simulink library "outp"  (R2021b)
(part 11 of 11)

  VSYS_PmicBootPath_raw32_Inproc/1 -> UnitConverter707/1
  UnitConverter707/1 -> VOUTP_PmicBootPath_raw32/1  "VOUTP_PmicBootPath_raw32"
  VSYS_DrivingMode_cnt/1 -> VSYS_DrivingMode_cnt_Inproc/1  "VSYS_DrivingMode_cnt"
  VSYS_DrivingMode_cnt_Inproc/1 -> UnitConverter708/1
  UnitConverter708/1 -> VOUTP_DrivingMode_cnt/1  "VOUTP_DrivingMode_cnt"
  VSYS_ModelYear_cnt/1 -> VSYS_ModelYear_cnt_Inproc/1  "VSYS_ModelYear_cnt"
  VSYS_ModelYear_cnt_Inproc/1 -> UnitConverter709/1
  UnitConverter709/1 -> VOUTP_ModelYear_cnt/1  "VOUTP_ModelYear_cnt"
  VSYS_Var4_cnt/1 -> VSYS_Var4_cnt_Inproc/1  "VSYS_Var4_cnt"
  VSYS_Var4_cnt_Inproc/1 -> UnitConverter710/1
  UnitConverter710/1 -> VOUTP_Var4_cnt/1  "VOUTP_Var4_cnt"
  VSYS_Var5_cnt/1 -> VSYS_Var5_cnt_Inproc/1  "VSYS_Var5_cnt"
  VSYS_Var5_cnt_Inproc/1 -> UnitConverter711/1
  UnitConverter711/1 -> VOUTP_Var5_cnt/1  "VOUTP_Var5_cnt"
  VTHC_FDCompCmd_rpm/1 -> VTHC_FDCompCmd_rpm_Inproc/1  "VTHC_FDCompCmd_rpm"
  VTHC_FDCompCmd_rpm_Inproc/1 -> UnitConverter712/1
  UnitConverter712/1 -> VOUTP_FDCompCmd_rpm/1  "VOUTP_FDCompCmd_rpm"
  VTHC_FDSOV1Cmd_flg/1 -> VTHC_FDSOV1Cmd_flg_Inproc/1  "VTHC_FDSOV1Cmd_flg"
  VTHC_FDSOV1Cmd_flg_Inproc/1 -> UnitConverter713/1
  UnitConverter713/1 -> VOUTP_FDSOV1Cmd_flg/1  "VOUTP_FDSOV1Cmd_flg"
  VTHC_FDSOV2Cmd_flg/1 -> VTHC_FDSOV2Cmd_flg_Inproc/1  "VTHC_FDSOV2Cmd_flg"
  VTHC_FDSOV2Cmd_flg_Inproc/1 -> UnitConverter714/1
  UnitConverter714/1 -> VOUTP_FDSOV2Cmd_flg/1  "VOUTP_FDSOV2Cmd_flg"
  VTHC_FDSOV3Cmd_flg/1 -> VTHC_FDSOV3Cmd_flg_Inproc/1  "VTHC_FDSOV3Cmd_flg"
  VTHC_FDSOV3Cmd_flg_Inproc/1 -> UnitConverter715/1
  UnitConverter715/1 -> VOUTP_FDSOV3Cmd_flg/1  "VOUTP_FDSOV3Cmd_flg"
  VTHC_FDEXV1Cmd_step/1 -> VTHC_FDEXV1Cmd_step_Inproc/1  "VTHC_FDEXV1Cmd_step"
  VTHC_FDEXV1Cmd_step_Inproc/1 -> UnitConverter716/1
  UnitConverter716/1 -> VOUTP_FDEXV1Cmd_step/1  "VOUTP_FDEXV1Cmd_step"
  VTHC_FDEXV2Cmd_step/1 -> VTHC_FDEXV2Cmd_step_Inproc/1  "VTHC_FDEXV2Cmd_step"
  VTHC_FDEXV2Cmd_step_Inproc/1 -> UnitConverter717/1
  UnitConverter717/1 -> VOUTP_FDEXV2Cmd_step/1  "VOUTP_FDEXV2Cmd_step"
  VTHC_FDSOTXVCmd_flg/1 -> VTHC_FDSOTXVCmd_flg_Inproc/1  "VTHC_FDSOTXVCmd_flg"
  VTHC_FDSOTXVCmd_flg_Inproc/1 -> UnitConverter718/1
  UnitConverter718/1 -> VOUTP_FDSOTXVCmd_flg/1  "VOUTP_FDSOTXVCmd_flg"
  VTHC_FDFWVCmd_flg/1 -> VTHC_FDFWVCmd_flg_Inproc/1  "VTHC_FDFWVCmd_flg"
  VTHC_FDFWVCmd_flg_Inproc/1 -> UnitConverter719/1
  UnitConverter719/1 -> VOUTP_FDFWVCmd_flg/1  "VOUTP_FDFWVCmd_flg"
  VTHC_FDTWVCmd_pct/1 -> VTHC_FDTWVCmd_pct_Inproc/1  "VTHC_FDTWVCmd_pct"
  VTHC_FDTWVCmd_pct_Inproc/1 -> UnitConverter720/1
  UnitConverter720/1 -> VOUTP_FDTWVCmd_pct/1  "VOUTP_FDTWVCmd_pct"
  VTHC_FDFrWPTCHeatPwrCmd_W/1 -> VTHC_FDFrWPTCHeatPwrCmd_W_Inproc/1  "VTHC_FDFrWPTCHeatPwrCmd_W"
  VTHC_FDFrWPTCHeatPwrCmd_W_Inproc/1 -> UnitConverter721/1
  UnitConverter721/1 -> VOUTP_FDFrWPTCHeatPwrCmd_W/1  "VOUTP_FDFrWPTCHeatPwrCmd_W"
  VTHC_CoolgFanActDuty_pct/1 -> VTHC_CoolgFanActDuty_pct_Inproc/1  "VTHC_CoolgFanActDuty_pct"
  VTHC_CoolgFanActDuty_pct_Inproc/1 -> UnitConverter722/1
  UnitConverter722/1 -> VOUTP_CoolgFanActDuty_pct/1  "VOUTP_CoolgFanActDuty_pct"
  VTHC_FDAGSCmd_enum/1 -> VTHC_FDAGSCmd_enum_Inproc/1  "VTHC_FDAGSCmd_enum"
  VTHC_FDAGSCmd_enum_Inproc/1 -> UnitConverter723/1
  UnitConverter723/1 -> VOUTP_FDAGSCmd_enum/1  "VOUTP_FDAGSCmd_enum"
  VTHC_FDEWP1Cmd_enum/1 -> VTHC_FDEWP1Cmd_enum_Inproc/1  "VTHC_FDEWP1Cmd_enum"
  VTHC_FDEWP1Cmd_enum_Inproc/1 -> UnitConverter724/1
  UnitConverter724/1 -> VOUTP_FDEWP1Cmd_enum/1  "VOUTP_FDEWP1Cmd_enum"
  VTHC_FDEWP2Cmd_enum/1 -> VTHC_FDEWP2Cmd_enum_Inproc/1  "VTHC_FDEWP2Cmd_enum"
  VTHC_FDEWP2Cmd_enum_Inproc/1 -> UnitConverter725/1
  UnitConverter725/1 -> VOUTP_FDEWP2Cmd_enum/1  "VOUTP_FDEWP2Cmd_enum"
  VTHC_FDEWP3Cmd_enum/1 -> VTHC_FDEWP3Cmd_enum_Inproc/1  "VTHC_FDEWP3Cmd_enum"
  VTHC_FDEWP3Cmd_enum_Inproc/1 -> UnitConverter726/1
  UnitConverter726/1 -> VOUTP_FDEWP3Cmd_enum/1  "VOUTP_FDEWP3Cmd_enum"
  VTHC_FDFrLeAPTCHeatPwrCmd_W/1 -> VTHC_FDFrLeAPTCHeatPwrCmd_W_Inproc/1  "VTHC_FDFrLeAPTCHeatPwrCmd_W"
  VTHC_FDFrLeAPTCHeatPwrCmd_W_Inproc/1 -> UnitConverter727/1
  UnitConverter727/1 -> VOUTP_FDFrLeAPTCHeatPwrCmd_W/1  "VOUTP_FDFrLeAPTCHeatPwrCmd_W"
  VTHC_FDFrRiAPTCHeatPwrCmd_W/1 -> VTHC_FDFrRiAPTCHeatPwrCmd_W_Inproc/1  "VTHC_FDFrRiAPTCHeatPwrCmd_W"
  VTHC_FDFrRiAPTCHeatPwrCmd_W_Inproc/1 -> UnitConverter728/1
  UnitConverter728/1 -> VOUTP_FDFrRiAPTCHeatPwrCmd_W/1  "VOUTP_FDFrRiAPTCHeatPwrCmd_W"
  VTHC_FDRrAPTCHeatPwrCmd_W/1 -> VTHC_FDRrAPTCHeatPwrCmd_W_Inproc/1  "VTHC_FDRrAPTCHeatPwrCmd_W"
  VTHC_FDRrAPTCHeatPwrCmd_W_Inproc/1 -> UnitConverter729/1
  UnitConverter729/1 -> VOUTP_FDRrAPTCHeatPwrCmd_W/1  "VOUTP_FDRrAPTCHeatPwrCmd_W"
  VTHC_FDBlowerCmd_pct/1 -> VTHC_FDBlowerCmd_pct_Inproc/1  "VTHC_FDBlowerCmd_pct"
  VTHC_FDBlowerCmd_pct_Inproc/1 -> UnitConverter730/1
  UnitConverter730/1 -> VOUTP_FDBlowerCmd_pct/1  "VOUTP_FDBlowerCmd_pct"
  VTHC_BatteryMode_enum/1 -> VTHC_BatteryMode_enum_Inproc/1  "VTHC_BatteryMode_enum"
  VTHC_BatteryMode_enum_Inproc/1 -> UnitConverter731/1
  UnitConverter731/1 -> VOUTP_BatteryMode_enum/1  "VOUTP_BatteryMode_enum"
  VTHC_EDriveMode_enum/1 -> VTHC_EDriveMode_enum_Inproc/1  "VTHC_EDriveMode_enum"
  VTHC_EDriveMode_enum_Inproc/1 -> UnitConverter732/1
  UnitConverter732/1 -> VOUTP_EDriveMode_enum/1  "VOUTP_EDriveMode_enum"
  VTHC_CabinMode_enum/1 -> VTHC_CabinMode_enum_Inproc/1  "VTHC_CabinMode_enum"
  VTHC_CabinMode_enum_Inproc/1 -> UnitConverter733/1
  UnitConverter733/1 -> VOUTP_CabinMode_enum/1  "VOUTP_CabinMode_enum"
  VTHC_CCUACLampSts_flg/1 -> VTHC_CCUACLampSts_flg_Inproc/1  "VTHC_CCUACLampSts_flg"
  VTHC_CCUACLampSts_flg_Inproc/1 -> UnitConverter734/1
  UnitConverter734/1 -> VOUTP_CCUACLampSts_flg/1  "VOUTP_CCUACLampSts_flg"
  VTHC_CCUAutoLampSts_flg/1 -> VTHC_CCUAutoLampSts_flg_Inproc/1  "VTHC_CCUAutoLampSts_flg"
  VTHC_CCUAutoLampSts_flg_Inproc/1 -> UnitConverter735/1
  UnitConverter735/1 -> VOUTP_CCUAutoLampSts_flg/1  "VOUTP_CCUAutoLampSts_flg"
  VTHC_CCUACMaxLampSts_flg/1 -> VTHC_CCUACMaxLampSts_flg_Inproc/1  "VTHC_CCUACMaxLampSts_flg"
  VTHC_CCUACMaxLampSts_flg_Inproc/1 -> UnitConverter736/1
  UnitConverter736/1 -> VOUTP_CCUACMaxLampSts_flg/1  "VOUTP_CCUACMaxLampSts_flg"
  VTHC_CCUSyncLampSts_flg/1 -> VTHC_CCUSyncLampSts_flg_Inproc/1  "VTHC_CCUSyncLampSts_flg"
  VTHC_CCUSyncLampSts_flg_Inproc/1 -> UnitConverter737/1
  UnitConverter737/1 -> VOUTP_CCUSyncLampSts_flg/1  "VOUTP_CCUSyncLampSts_flg"
  VTHC_sigAirIntenZon1St_enum/1 -> VTHC_sigAirIntenZon1St_enum_Inproc/1  "VTHC_sigAirIntenZon1St_enum"
  VTHC_sigAirIntenZon1St_enum_Inproc/1 -> UnitConverter738/1
  UnitConverter738/1 -> VOUTP_sigAirIntenZon1St_enum/1  "VOUTP_sigAirIntenZon1St_enum"
  VTHC_sigWindDirZon1St_enum/1 -> VTHC_sigWindDirZon1St_enum_Inproc/1  "VTHC_sigWindDirZon1St_enum"
  VTHC_sigWindDirZon1St_enum_Inproc/1 -> UnitConverter739/1
  UnitConverter739/1 -> VOUTP_sigWindDirZon1St_enum/1  "VOUTP_sigWindDirZon1St_enum"
  VTHC_sigRecircSt_flg/1 -> VTHC_sigRecircSt_flg_Inproc/1  "VTHC_sigRecircSt_flg"
  VTHC_sigRecircSt_flg_Inproc/1 -> UnitConverter740/1
  UnitConverter740/1 -> VOUTP_sigRecircSt_flg/1  "VOUTP_sigRecircSt_flg"
  VTHC_sigSetTempZon1St_C/1 -> VTHC_sigSetTempZon1St_C_Inproc/1  "VTHC_sigSetTempZon1St_C"
  VTHC_sigSetTempZon1St_C_Inproc/1 -> UnitConverter741/1
  UnitConverter741/1 -> VOUTP_sigSetTempZon1St_C/1  "VOUTP_sigSetTempZon1St_C"
  VTHC_sigSetTempZon2St_C/1 -> VTHC_sigSetTempZon2St_C_Inproc/1  "VTHC_sigSetTempZon2St_C"
  VTHC_sigSetTempZon2St_C_Inproc/1 -> UnitConverter742/1
  UnitConverter742/1 -> VOUTP_sigSetTempZon2St_C/1  "VOUTP_sigSetTempZon2St_C"
  VTHC_sigClntTHvBattOut_C/1 -> VTHC_sigClntTHvBattOut_C_Inproc/1  "VTHC_sigClntTHvBattOut_C"
  VTHC_sigClntTHvBattOut_C_Inproc/1 -> UnitConverter743/1
  UnitConverter743/1 -> VOUTP_sigClntTHvBattOut_C/1  "VOUTP_sigClntTHvBattOut_C"
  VTHC_sigCbnSolarLeft_W/1 -> VTHC_sigCbnSolarLeft_W_Inproc/1  "VTHC_sigCbnSolarLeft_W"
  VTHC_sigCbnSolarLeft_W_Inproc/1 -> UnitConverter744/1
  UnitConverter744/1 -> VOUTP_sigCbnSolarLeft_W/1  "VOUTP_sigCbnSolarLeft_W"
  VTHC_sigClntTHvBattIn_C/1 -> VTHC_sigClntTHvBattIn_C_Inproc/1  "VTHC_sigClntTHvBattIn_C"
  VTHC_sigClntTHvBattIn_C_Inproc/1 -> UnitConverter745/1
  UnitConverter745/1 -> VOUTP_sigClntTHvBattIn_C/1  "VOUTP_sigClntTHvBattIn_C"
  VTHC_sigCbnSolarRight_W/1 -> VTHC_sigCbnSolarRight_W_Inproc/1  "VTHC_sigCbnSolarRight_W"
  VTHC_sigCbnSolarRight_W_Inproc/1 -> UnitConverter746/1
  UnitConverter746/1 -> VOUTP_sigCbnSolarRight_W/1  "VOUTP_sigCbnSolarRight_W"
  VTHC_sigAmbAirT_C/1 -> VTHC_sigAmbAirT_C_Inproc/1  "VTHC_sigAmbAirT_C"
  VTHC_sigAmbAirT_C_Inproc/1 -> UnitConverter747/1
  UnitConverter747/1 -> VOUTP_sigAmbAirT_C/1  "VOUTP_sigAmbAirT_C"
  VTHC_sigCbnAirT_C/1 -> VTHC_sigCbnAirT_C_Inproc/1  "VTHC_sigCbnAirT_C"
  VTHC_sigCbnAirT_C_Inproc/1 -> UnitConverter748/1
  UnitConverter748/1 -> VOUTP_sigCbnAirT_C/1  "VOUTP_sigCbnAirT_C"
  VTHC_ACSubMode_enum/1 -> VTHC_ACSubMode_enum_Inproc/1  "VTHC_ACSubMode_enum"
  VTHC_ACSubMode_enum_Inproc/1 -> UnitConverter749/1
  UnitConverter749/1 -> VOUTP_ACSubMode_enum/1  "VOUTP_ACSubMode_enum"
  VTHC_FDRecyAutoCmd_enum/1 -> VTHC_FDRecyAutoCmd_enum_Inproc/1  "VTHC_FDRecyAutoCmd_enum"
  VTHC_FDRecyAutoCmd_enum_Inproc/1 -> UnitConverter750/1
  UnitConverter750/1 -> VOUTP_FDRecyAutoCmd_enum/1  "VOUTP_FDRecyAutoCmd_enum"
  VTHC_ACModeMem_enum/1 -> VTHC_ACModeMem_enum_Inproc/1  "VTHC_ACModeMem_enum"
  VTHC_ACModeMem_enum_Inproc/1 -> UnitConverter751/1
  UnitConverter751/1 -> VOUTP_ACModeMem_enum/1  "VOUTP_ACModeMem_enum"
  VTHC_Face_flg/1 -> VTHC_Face_flg_Inproc/1  "VTHC_Face_flg"
  VTHC_Face_flg_Inproc/1 -> UnitConverter752/1
  UnitConverter752/1 -> VOUTP_Face_flg/1  "VOUTP_Face_flg"
  VTHC_Foot_flg/1 -> VTHC_Foot_flg_Inproc/1  "VTHC_Foot_flg"
  VTHC_Foot_flg_Inproc/1 -> UnitConverter753/1
  UnitConverter753/1 -> VOUTP_Foot_flg/1  "VOUTP_Foot_flg"
  VTHC_Frost_flg/1 -> VTHC_Frost_flg_Inproc/1  "VTHC_Frost_flg"
  VTHC_Frost_flg_Inproc/1 -> UnitConverter754/1
  UnitConverter754/1 -> VOUTP_Frost_flg/1  "VOUTP_Frost_flg"
  VTHC_FaceM_flg/1 -> VTHC_FaceM_flg_Inproc/1  "VTHC_FaceM_flg"
  VTHC_FaceM_flg_Inproc/1 -> UnitConverter755/1
  UnitConverter755/1 -> VOUTP_FaceM_flg/1  "VOUTP_FaceM_flg"
  VTHC_FootM_flg/1 -> VTHC_FootM_flg_Inproc/1  "VTHC_FootM_flg"
  VTHC_FootM_flg_Inproc/1 -> UnitConverter756/1
  UnitConverter756/1 -> VOUTP_FootM_flg/1  "VOUTP_FootM_flg"
  VTHC_CCUSyncSts_flg/1 -> VTHC_CCUSyncSts_flg_Inproc/1  "VTHC_CCUSyncSts_flg"
  VTHC_CCUSyncSts_flg_Inproc/1 -> UnitConverter757/1
  UnitConverter757/1 -> VOUTP_CCUSyncSts_flg/1  "VOUTP_CCUSyncSts_flg"
  VTHC_ACForceOFF_flg/1 -> VTHC_ACForceOFF_flg_Inproc/1  "VTHC_ACForceOFF_flg"
  VTHC_ACForceOFF_flg_Inproc/1 -> UnitConverter758/1
  UnitConverter758/1 -> VOUTP_ACForceOFF_flg/1  "VOUTP_ACForceOFF_flg"
  VTHC_RecAutoFlg_flg/1 -> VTHC_RecAutoFlg_flg_Inproc/1  "VTHC_RecAutoFlg_flg"
  VTHC_RecAutoFlg_flg_Inproc/1 -> UnitConverter759/1
  UnitConverter759/1 -> VOUTP_RecAutoFlg_flg/1  "VOUTP_RecAutoFlg_flg"
  VTHC_AirIntenZone1M_enum/1 -> VTHC_AirIntenZone1M_enum_Inproc/1  "VTHC_AirIntenZone1M_enum"
  VTHC_AirIntenZone1M_enum_Inproc/1 -> UnitConverter760/1
  UnitConverter760/1 -> VOUTP_AirIntenZone1M_enum/1  "VOUTP_AirIntenZone1M_enum"
  VTHC_fdefog_flg/1 -> VTHC_fdefog_flg_Inproc/1  "VTHC_fdefog_flg"
  VTHC_fdefog_flg_Inproc/1 -> UnitConverter761/1
  UnitConverter761/1 -> VOUTP_fdefog_flg/1  "VOUTP_fdefog_flg"
  VTHC_sigSetTempZon2StM_C/1 -> VTHC_sigSetTempZon2StM_C_Inproc/1  "VTHC_sigSetTempZon2StM_C"
  VTHC_sigSetTempZon2StM_C_Inproc/1 -> UnitConverter762/1
  UnitConverter762/1 -> VOUTP_sigSetTempZon2StM_C/1  "VOUTP_sigSetTempZon2StM_C"
  VTHC_sigDfrstSt_flg/1 -> VTHC_sigDfrstSt_flg_Inproc/1  "VTHC_sigDfrstSt_flg"
  VTHC_sigDfrstSt_flg_Inproc/1 -> UnitConverter763/1
  UnitConverter763/1 -> VOUTP_sigDfrstSt_flg/1  "VOUTP_sigDfrstSt_flg"
  VTHC_FDCTHCAirIntZ3Sta_enum/1 -> VTHC_FDCTHCAirIntZ3Sta_enum_Inproc/1  "VTHC_FDCTHCAirIntZ3Sta_enum"
  VTHC_FDCTHCAirIntZ3Sta_enum_Inproc/1 -> UnitConverter764/1
  UnitConverter764/1 -> VOUTP_FDCTHCAirIntZ3Sta_enum/1  "VOUTP_FDCTHCAirIntZ3Sta_enum"
  VTHC_FDCTHCLEVentModeSta_enum/1 -> VTHC_FDCTHCLEVentModeSta_enum_Inproc/1  "VTHC_FDCTHCLEVentModeSta_enum"
  VTHC_FDCTHCLEVentModeSta_enum_Inproc/1 -> UnitConverter765/1
  UnitConverter765/1 -> VOUTP_FDCTHCLEVentModeSta_enum/1  "VOUTP_FDCTHCLEVentModeSta_enum"
  VTHC_FDCTHCREVentModeSta_enum/1 -> VTHC_FDCTHCREVentModeSta_enum_Inproc/1  "VTHC_FDCTHCREVentModeSta_enum"
  VTHC_FDCTHCREVentModeSta_enum_Inproc/1 -> UnitConverter766/1
  UnitConverter766/1 -> VOUTP_FDCTHCREVentModeSta_enum/1  "VOUTP_FDCTHCREVentModeSta_enum"
  VTHC_FDCTHCLEVentZSta_enum/1 -> VTHC_FDCTHCLEVentZSta_enum_Inproc/1  "VTHC_FDCTHCLEVentZSta_enum"
  VTHC_FDCTHCLEVentZSta_enum_Inproc/1 -> UnitConverter767/1
  UnitConverter767/1 -> VOUTP_FDCTHCLEVentZSta_enum/1  "VOUTP_FDCTHCLEVentZSta_enum"
  VTHC_FDCTHCCLEVentZSta_enum/1 -> VTHC_FDCTHCCLEVentZSta_enum_Inproc/1  "VTHC_FDCTHCCLEVentZSta_enum"
  VTHC_FDCTHCCLEVentZSta_enum_Inproc/1 -> UnitConverter768/1
  UnitConverter768/1 -> VOUTP_FDCTHCCLEVentZSta_enum/1  "VOUTP_FDCTHCCLEVentZSta_enum"
  VTHC_FDCTHCREVentZSta_enum/1 -> VTHC_FDCTHCREVentZSta_enum_Inproc/1  "VTHC_FDCTHCREVentZSta_enum"
  VTHC_FDCTHCREVentZSta_enum_Inproc/1 -> UnitConverter769/1
  UnitConverter769/1 -> VOUTP_FDCTHCREVentZSta_enum/1  "VOUTP_FDCTHCREVentZSta_enum"
  VTHC_FDCTHCCREVentZSta_enum/1 -> VTHC_FDCTHCCREVentZSta_enum_Inproc/1  "VTHC_FDCTHCCREVentZSta_enum"
  VTHC_FDCTHCCREVentZSta_enum_Inproc/1 -> UnitConverter770/1
  UnitConverter770/1 -> VOUTP_FDCTHCCREVentZSta_enum/1  "VOUTP_FDCTHCCREVentZSta_enum"
  VTHC_FDCTHCLEVentYSta_enum/1 -> VTHC_FDCTHCLEVentYSta_enum_Inproc/1  "VTHC_FDCTHCLEVentYSta_enum"
  VTHC_FDCTHCLEVentYSta_enum_Inproc/1 -> UnitConverter771/1
  UnitConverter771/1 -> VOUTP_FDCTHCLEVentYSta_enum/1  "VOUTP_FDCTHCLEVentYSta_enum"
  VTHC_FDCTHCLVentENSta_flg/1 -> VTHC_FDCTHCLVentENSta_flg_Inproc/1  "VTHC_FDCTHCLVentENSta_flg"
  VTHC_FDCTHCLVentENSta_flg_Inproc/1 -> UnitConverter772/1
  UnitConverter772/1 -> VOUTP_FDCTHCLVentENSta_flg/1  "VOUTP_FDCTHCLVentENSta_flg"
  VTHC_FDCTHCCLEVentYSta_enum/1 -> VTHC_FDCTHCCLEVentYSta_enum_Inproc/1  "VTHC_FDCTHCCLEVentYSta_enum"
  VTHC_FDCTHCCLEVentYSta_enum_Inproc/1 -> UnitConverter773/1
  UnitConverter773/1 -> VOUTP_FDCTHCCLEVentYSta_enum/1  "VOUTP_FDCTHCCLEVentYSta_enum"
  VTHC_FDCTHCCLVentENSta_flg/1 -> VTHC_FDCTHCCLVentENSta_flg_Inproc/1  "VTHC_FDCTHCCLVentENSta_flg"
  VTHC_FDCTHCCLVentENSta_flg_Inproc/1 -> UnitConverter774/1
  UnitConverter774/1 -> VOUTP_FDCTHCCLVentENSta_flg/1  "VOUTP_FDCTHCCLVentENSta_flg"
  VTHC_FDCTHCREVentYSta_enum/1 -> VTHC_FDCTHCREVentYSta_enum_Inproc/1  "VTHC_FDCTHCREVentYSta_enum"
  VTHC_FDCTHCREVentYSta_enum_Inproc/1 -> UnitConverter775/1
  UnitConverter775/1 -> VOUTP_FDCTHCREVentYSta_enum/1  "VOUTP_FDCTHCREVentYSta_enum"
  VTHC_FDCTHCRVentENSta_flg/1 -> VTHC_FDCTHCRVentENSta_flg_Inproc/1  "VTHC_FDCTHCRVentENSta_flg"
  VTHC_FDCTHCRVentENSta_flg_Inproc/1 -> UnitConverter776/1
  UnitConverter776/1 -> VOUTP_FDCTHCRVentENSta_flg/1  "VOUTP_FDCTHCRVentENSta_flg"
  VTHC_FDCTHCCREVentYSta_enum/1 -> VTHC_FDCTHCCREVentYSta_enum_Inproc/1  "VTHC_FDCTHCCREVentYSta_enum"
  VTHC_FDCTHCCREVentYSta_enum_Inproc/1 -> UnitConverter777/1
  UnitConverter777/1 -> VOUTP_FDCTHCCREVentYSta_enum/1  "VOUTP_FDCTHCCREVentYSta_enum"
  VTHC_FDCTHCCRVentENSta_flg/1 -> VTHC_FDCTHCCRVentENSta_flg_Inproc/1  "VTHC_FDCTHCCRVentENSta_flg"
  VTHC_FDCTHCCRVentENSta_flg_Inproc/1 -> UnitConverter778/1
  UnitConverter778/1 -> VOUTP_FDCTHCCRVentENSta_flg/1  "VOUTP_FDCTHCCRVentENSta_flg"
  VTHC_FDCTHCMAPTCForceOFFSta_flg/1 -> VTHC_FDCTHCMAPTCForceOFFSta_flg_Inproc/1  "VTHC_FDCTHCMAPTCForceOFFSta_flg"
  VTHC_FDCTHCMAPTCForceOFFSta_flg_Inproc/1 -> UnitConverter779/1
  UnitConverter779/1 -> VOUTP_FDCTHCMAPTCForceOFFSta_flg/1  "VOUTP_FDCTHCMAPTCForceOFFSta_flg"
  VTHC_FDCFGSAirIntSta_enum/1 -> VTHC_FDCFGSAirIntSta_enum_Inproc/1  "VTHC_FDCFGSAirIntSta_enum"
  VTHC_FDCFGSAirIntSta_enum_Inproc/1 -> UnitConverter780/1
  UnitConverter780/1 -> VOUTP_FDCFGSAirIntSta_enum/1  "VOUTP_FDCFGSAirIntSta_enum"
  VTHC_FDCFGSChSta_enum/1 -> VTHC_FDCFGSChSta_enum_Inproc/1  "VTHC_FDCFGSChSta_enum"
  VTHC_FDCFGSChSta_enum_Inproc/1 -> UnitConverter781/1
  UnitConverter781/1 -> VOUTP_FDCFGSChSta_enum/1  "VOUTP_FDCFGSChSta_enum"
  VTHC_FDCFGSAirIntCmd_enum/1 -> VTHC_FDCFGSAirIntCmd_enum_Inproc/1  "VTHC_FDCFGSAirIntCmd_enum"
  VTHC_FDCFGSAirIntCmd_enum_Inproc/1 -> UnitConverter782/1
  UnitConverter782/1 -> VOUTP_FDCFGSAirIntCmd_enum/1  "VOUTP_FDCFGSAirIntCmd_enum"
  VTHC_FDCFGSFuncSta_enum/1 -> VTHC_FDCFGSFuncSta_enum_Inproc/1  "VTHC_FDCFGSFuncSta_enum"
  VTHC_FDCFGSFuncSta_enum_Inproc/1 -> UnitConverter783/1
  UnitConverter783/1 -> VOUTP_FDCFGSFuncSta_enum/1  "VOUTP_FDCFGSFuncSta_enum"
  VTHC_FDCFGSChCmd_enum/1 -> VTHC_FDCFGSChCmd_enum_Inproc/1  "VTHC_FDCFGSChCmd_enum"
  VTHC_FDCFGSChCmd_enum_Inproc/1 -> UnitConverter784/1
  UnitConverter784/1 -> VOUTP_FDCFGSChCmd_enum/1  "VOUTP_FDCFGSChCmd_enum"
  VTHC_FDCFGSIONSWSta_flg/1 -> VTHC_FDCFGSIONSWSta_flg_Inproc/1  "VTHC_FDCFGSIONSWSta_flg"
  VTHC_FDCFGSIONSWSta_flg_Inproc/1 -> UnitConverter785/1
  UnitConverter785/1 -> VOUTP_FDCFGSIONSWSta_flg/1  "VOUTP_FDCFGSIONSWSta_flg"
  VTHC_FDCFGSIONCmd_flg/1 -> VTHC_FDCFGSIONCmd_flg_Inproc/1  "VTHC_FDCFGSIONCmd_flg"
  VTHC_FDCFGSIONCmd_flg_Inproc/1 -> UnitConverter786/1
  UnitConverter786/1 -> VOUTP_FDCFGSIONCmd_flg/1  "VOUTP_FDCFGSIONCmd_flg"
  VTHC_FDCTHCMPreWPTCHeatSta_enum/1 -> VTHC_FDCTHCMPreWPTCHeatSta_enum_Inproc/1  "VTHC_FDCTHCMPreWPTCHeatSta_enum"
  VTHC_FDCTHCMPreWPTCHeatSta_enum_Inproc/1 -> UnitConverter787/1
  UnitConverter787/1 -> VOUTP_FDCTHCMPreWPTCHeatSta_enum/1  "VOUTP_FDCTHCMPreWPTCHeatSta_enum"
  VTHC_EWPBUflag1_flg/1 -> VTHC_EWPBUflag1_flg_Inproc/1  "VTHC_EWPBUflag1_flg"
  VTHC_EWPBUflag1_flg_Inproc/1 -> UnitConverter788/1
  UnitConverter788/1 -> VOUTP_EWPBUflag1_flg/1  "VOUTP_EWPBUflag1_flg"
  VTHC_EWPBUflag2_flg/1 -> VTHC_EWPBUflag2_flg_Inproc/1  "VTHC_EWPBUflag2_flg"
  VTHC_EWPBUflag2_flg_Inproc/1 -> UnitConverter789/1
  UnitConverter789/1 -> VOUTP_EWPBUflag2_flg/1  "VOUTP_EWPBUflag2_flg"
  VTHC_EWPBUflag3_flg/1 -> VTHC_EWPBUflag3_flg_Inproc/1  "VTHC_EWPBUflag3_flg"
  VTHC_EWPBUflag3_flg_Inproc/1 -> UnitConverter790/1
  UnitConverter790/1 -> VOUTP_EWPBUflag3_flg/1  "VOUTP_EWPBUflag3_flg"
  VTHC_FaceMSet_enum/1 -> VTHC_FaceMSet_enum_Inproc/1  "VTHC_FaceMSet_enum"
  VTHC_FaceMSet_enum_Inproc/1 -> UnitConverter791/1
  UnitConverter791/1 -> VOUTP_FaceMSet_enum/1  "VOUTP_FaceMSet_enum"
  VTHC_FootMSet_enum/1 -> VTHC_FootMSet_enum_Inproc/1  "VTHC_FootMSet_enum"
  VTHC_FootMSet_enum_Inproc/1 -> UnitConverter792/1
  UnitConverter792/1 -> VOUTP_FootMSet_enum/1  "VOUTP_FootMSet_enum"
  VTHC_fdefogSet_enum/1 -> VTHC_fdefogSet_enum_Inproc/1  "VTHC_fdefogSet_enum"
  VTHC_fdefogSet_enum_Inproc/1 -> UnitConverter793/1
  UnitConverter793/1 -> VOUTP_fdefogSet_enum/1  "VOUTP_fdefogSet_enum"
  VTHC_CCUSyncStsSet_enum/1 -> VTHC_CCUSyncStsSet_enum_Inproc/1  "VTHC_CCUSyncStsSet_enum"
  VTHC_CCUSyncStsSet_enum_Inproc/1 -> UnitConverter794/1
  UnitConverter794/1 -> VOUTP_CCUSyncStsSet_enum/1  "VOUTP_CCUSyncStsSet_enum"
  VTHC_sigRecircStSet_enum/1 -> VTHC_sigRecircStSet_enum_Inproc/1  "VTHC_sigRecircStSet_enum"
  VTHC_sigRecircStSet_enum_Inproc/1 -> UnitConverter795/1
  UnitConverter795/1 -> VOUTP_sigRecircStSet_enum/1  "VOUTP_sigRecircStSet_enum"
  VTHC_RecyAutoSet_enum/1 -> VTHC_RecyAutoSet_enum_Inproc/1  "VTHC_RecyAutoSet_enum"
  VTHC_RecyAutoSet_enum_Inproc/1 -> UnitConverter796/1
  UnitConverter796/1 -> VOUTP_RecyAutoSet_enum/1  "VOUTP_RecyAutoSet_enum"
  VTHC_AirIntenZone1MSet1_enum/1 -> VTHC_AirIntenZone1MSet1_enum_Inproc/1  "VTHC_AirIntenZone1MSet1_enum"
  VTHC_AirIntenZone1MSet1_enum_Inproc/1 -> UnitConverter797/1
  UnitConverter797/1 -> VOUTP_AirIntenZone1MSet1_enum/1  "VOUTP_AirIntenZone1MSet1_enum"
  VTHC_AirIntenZone1MSet2_enum/1 -> VTHC_AirIntenZone1MSet2_enum_Inproc/1  "VTHC_AirIntenZone1MSet2_enum"
  VTHC_AirIntenZone1MSet2_enum_Inproc/1 -> UnitConverter798/1
  UnitConverter798/1 -> VOUTP_AirIntenZone1MSet2_enum/1  "VOUTP_AirIntenZone1MSet2_enum"
  VTHC_AirIntenZone1MSet3_enum/1 -> VTHC_AirIntenZone1MSet3_enum_Inproc/1  "VTHC_AirIntenZone1MSet3_enum"
  VTHC_AirIntenZone1MSet3_enum_Inproc/1 -> UnitConverter799/1
  UnitConverter799/1 -> VOUTP_AirIntenZone1MSet3_enum/1  "VOUTP_AirIntenZone1MSet3_enum"
  VTHC_AirIntenZone1MSet4_enum/1 -> VTHC_AirIntenZone1MSet4_enum_Inproc/1  "VTHC_AirIntenZone1MSet4_enum"
  VTHC_AirIntenZone1MSet4_enum_Inproc/1 -> UnitConverter800/1
  UnitConverter800/1 -> VOUTP_AirIntenZone1MSet4_enum/1  "VOUTP_AirIntenZone1MSet4_enum"
  VTHC_AirIntenZone1MSet5_enum/1 -> VTHC_AirIntenZone1MSet5_enum_Inproc/1  "VTHC_AirIntenZone1MSet5_enum"
  VTHC_AirIntenZone1MSet5_enum_Inproc/1 -> UnitConverter801/1
  UnitConverter801/1 -> VOUTP_AirIntenZone1MSet5_enum/1  "VOUTP_AirIntenZone1MSet5_enum"
  VTHC_AirIntenZone1MSet7_enum/1 -> VTHC_AirIntenZone1MSet7_enum_Inproc/1  "VTHC_AirIntenZone1MSet7_enum"
  VTHC_AirIntenZone1MSet7_enum_Inproc/1 -> UnitConverter802/1
  UnitConverter802/1 -> VOUTP_AirIntenZone1MSet7_enum/1  "VOUTP_AirIntenZone1MSet7_enum"
  VTHC_AirIntenZone3MSet1_enum/1 -> VTHC_AirIntenZone3MSet1_enum_Inproc/1  "VTHC_AirIntenZone3MSet1_enum"
  VTHC_AirIntenZone3MSet1_enum_Inproc/1 -> UnitConverter803/1
  UnitConverter803/1 -> VOUTP_AirIntenZone3MSet1_enum/1  "VOUTP_AirIntenZone3MSet1_enum"
  VTHC_AirIntenZone3MSet2_enum/1 -> VTHC_AirIntenZone3MSet2_enum_Inproc/1  "VTHC_AirIntenZone3MSet2_enum"
  VTHC_AirIntenZone3MSet2_enum_Inproc/1 -> UnitConverter804/1
  UnitConverter804/1 -> VOUTP_AirIntenZone3MSet2_enum/1  "VOUTP_AirIntenZone3MSet2_enum"
  VTHC_AirIntenZone3MSet3_enum/1 -> VTHC_AirIntenZone3MSet3_enum_Inproc/1  "VTHC_AirIntenZone3MSet3_enum"
  VTHC_AirIntenZone3MSet3_enum_Inproc/1 -> UnitConverter805/1
  UnitConverter805/1 -> VOUTP_AirIntenZone3MSet3_enum/1  "VOUTP_AirIntenZone3MSet3_enum"
  VTHC_AirIntenZone3MSet4_enum/1 -> VTHC_AirIntenZone3MSet4_enum_Inproc/1  "VTHC_AirIntenZone3MSet4_enum"
  VTHC_AirIntenZone3MSet4_enum_Inproc/1 -> UnitConverter806/1
  UnitConverter806/1 -> VOUTP_AirIntenZone3MSet4_enum/1  "VOUTP_AirIntenZone3MSet4_enum"
  VTHC_AirIntenZone3MSet5_enum/1 -> VTHC_AirIntenZone3MSet5_enum_Inproc/1  "VTHC_AirIntenZone3MSet5_enum"
  VTHC_AirIntenZone3MSet5_enum_Inproc/1 -> UnitConverter807/1
  UnitConverter807/1 -> VOUTP_AirIntenZone3MSet5_enum/1  "VOUTP_AirIntenZone3MSet5_enum"
  VTHC_AirIntenZone3MSet7_enum/1 -> VTHC_AirIntenZone3MSet7_enum_Inproc/1  "VTHC_AirIntenZone3MSet7_enum"
  VTHC_AirIntenZone3MSet7_enum_Inproc/1 -> UnitConverter808/1
  UnitConverter808/1 -> VOUTP_AirIntenZone3MSet7_enum/1  "VOUTP_AirIntenZone3MSet7_enum"
  VTHC_IONSWStaSet_enum/1 -> VTHC_IONSWStaSet_enum_Inproc/1  "VTHC_IONSWStaSet_enum"
  VTHC_IONSWStaSet_enum_Inproc/1 -> UnitConverter809/1
  UnitConverter809/1 -> VOUTP_IONSWStaSet_enum/1  "VOUTP_IONSWStaSet_enum"
  VTHC_FDCFGSChStaSet123_enum/1 -> VTHC_FDCFGSChStaSet123_enum_Inproc/1  "VTHC_FDCFGSChStaSet123_enum"
  VTHC_FDCFGSChStaSet123_enum_Inproc/1 -> UnitConverter810/1
  UnitConverter810/1 -> VOUTP_FDCFGSChStaSet123_enum/1  "VOUTP_FDCFGSChStaSet123_enum"
  VTHC_FDCFGSChStaSet457_enum/1 -> VTHC_FDCFGSChStaSet457_enum_Inproc/1  "VTHC_FDCFGSChStaSet457_enum"
  VTHC_FDCFGSChStaSet457_enum_Inproc/1 -> UnitConverter811/1
  UnitConverter811/1 -> VOUTP_FDCFGSChStaSet457_enum/1  "VOUTP_FDCFGSChStaSet457_enum"
  VTHC_FDCFGSAirIntStaSet123_enum/1 -> VTHC_FDCFGSAirIntStaSet123_enum_Inproc/1  "VTHC_FDCFGSAirIntStaSet123_enum"
  VTHC_FDCFGSAirIntStaSet123_enum_Inproc/1 -> UnitConverter812/1
  UnitConverter812/1 -> VOUTP_FDCFGSAirIntStaSet123_enum/1  "VOUTP_FDCFGSAirIntStaSet123_enum"
  VTHC_FDCFGSAirIntStaSet457_enum/1 -> VTHC_FDCFGSAirIntStaSet457_enum_Inproc/1  "VTHC_FDCFGSAirIntStaSet457_enum"
  VTHC_FDCFGSAirIntStaSet457_enum_Inproc/1 -> UnitConverter813/1
  UnitConverter813/1 -> VOUTP_FDCFGSAirIntStaSet457_enum/1  "VOUTP_FDCFGSAirIntStaSet457_enum"
  VTHC_LVentENSet_enum/1 -> VTHC_LVentENSet_enum_Inproc/1  "VTHC_LVentENSet_enum"
  VTHC_LVentENSet_enum_Inproc/1 -> UnitConverter814/1
  UnitConverter814/1 -> VOUTP_LVentENSet_enum/1  "VOUTP_LVentENSet_enum"
  VTHC_CLVentENSet_enum/1 -> VTHC_CLVentENSet_enum_Inproc/1  "VTHC_CLVentENSet_enum"
  VTHC_CLVentENSet_enum_Inproc/1 -> UnitConverter815/1
  UnitConverter815/1 -> VOUTP_CLVentENSet_enum/1  "VOUTP_CLVentENSet_enum"
  VTHC_RVentENSet_enum/1 -> VTHC_RVentENSet_enum_Inproc/1  "VTHC_RVentENSet_enum"
  VTHC_RVentENSet_enum_Inproc/1 -> UnitConverter816/1
  UnitConverter816/1 -> VOUTP_RVentENSet_enum/1  "VOUTP_RVentENSet_enum"
  VTHC_CRVentENSet_enum/1 -> VTHC_CRVentENSet_enum_Inproc/1  "VTHC_CRVentENSet_enum"
  VTHC_CRVentENSet_enum_Inproc/1 -> UnitConverter817/1
  UnitConverter817/1 -> VOUTP_CRVentENSet_enum/1  "VOUTP_CRVentENSet_enum"
  VTHC_LEVentModeStaSet123_enum/1 -> VTHC_LEVentModeStaSet123_enum_Inproc/1  "VTHC_LEVentModeStaSet123_enum"
  VTHC_LEVentModeStaSet123_enum_Inproc/1 -> UnitConverter818/1
  UnitConverter818/1 -> VOUTP_LEVentModeStaSet123_enum/1  "VOUTP_LEVentModeStaSet123_enum"
  VTHC_LEVentModeStaSet457_enum/1 -> VTHC_LEVentModeStaSet457_enum_Inproc/1  "VTHC_LEVentModeStaSet457_enum"
  VTHC_LEVentModeStaSet457_enum_Inproc/1 -> UnitConverter819/1
  UnitConverter819/1 -> VOUTP_LEVentModeStaSet457_enum/1  "VOUTP_LEVentModeStaSet457_enum"
  VTHC_REVentModeStaSet123_enum/1 -> VTHC_REVentModeStaSet123_enum_Inproc/1  "VTHC_REVentModeStaSet123_enum"
  VTHC_REVentModeStaSet123_enum_Inproc/1 -> UnitConverter820/1
  UnitConverter820/1 -> VOUTP_REVentModeStaSet123_enum/1  "VOUTP_REVentModeStaSet123_enum"
  VTHC_REVentModeStaSet457_enum/1 -> VTHC_REVentModeStaSet457_enum_Inproc/1  "VTHC_REVentModeStaSet457_enum"
  VTHC_REVentModeStaSet457_enum_Inproc/1 -> UnitConverter821/1
  UnitConverter821/1 -> VOUTP_REVentModeStaSet457_enum/1  "VOUTP_REVentModeStaSet457_enum"
  VTHC_FDCTHCLEVentZStaSet1_enum/1 -> VTHC_FDCTHCLEVentZStaSet1_enum_Inproc/1  "VTHC_FDCTHCLEVentZStaSet1_enum"
  VTHC_FDCTHCLEVentZStaSet1_enum_Inproc/1 -> UnitConverter822/1
  UnitConverter822/1 -> VOUTP_FDCTHCLEVentZStaSet1_enum/1  "VOUTP_FDCTHCLEVentZStaSet1_enum"
  VTHC_FDCTHCLEVentZStaSet2_enum/1 -> VTHC_FDCTHCLEVentZStaSet2_enum_Inproc/1  "VTHC_FDCTHCLEVentZStaSet2_enum"
  VTHC_FDCTHCLEVentZStaSet2_enum_Inproc/1 -> UnitConverter823/1
  UnitConverter823/1 -> VOUTP_FDCTHCLEVentZStaSet2_enum/1  "VOUTP_FDCTHCLEVentZStaSet2_enum"
  VTHC_FDCTHCLEVentZStaSet3_enum/1 -> VTHC_FDCTHCLEVentZStaSet3_enum_Inproc/1  "VTHC_FDCTHCLEVentZStaSet3_enum"
  VTHC_FDCTHCLEVentZStaSet3_enum_Inproc/1 -> UnitConverter824/1
  UnitConverter824/1 -> VOUTP_FDCTHCLEVentZStaSet3_enum/1  "VOUTP_FDCTHCLEVentZStaSet3_enum"
  VTHC_FDCTHCLEVentZStaSet4_enum/1 -> VTHC_FDCTHCLEVentZStaSet4_enum_Inproc/1  "VTHC_FDCTHCLEVentZStaSet4_enum"
  VTHC_FDCTHCLEVentZStaSet4_enum_Inproc/1 -> UnitConverter825/1
  UnitConverter825/1 -> VOUTP_FDCTHCLEVentZStaSet4_enum/1  "VOUTP_FDCTHCLEVentZStaSet4_enum"
  VTHC_FDCTHCLEVentZStaSet5_enum/1 -> VTHC_FDCTHCLEVentZStaSet5_enum_Inproc/1  "VTHC_FDCTHCLEVentZStaSet5_enum"
  VTHC_FDCTHCLEVentZStaSet5_enum_Inproc/1 -> UnitConverter826/1
  UnitConverter826/1 -> VOUTP_FDCTHCLEVentZStaSet5_enum/1  "VOUTP_FDCTHCLEVentZStaSet5_enum"
  VTHC_FDCTHCLEVentZStaSet7_enum/1 -> VTHC_FDCTHCLEVentZStaSet7_enum_Inproc/1  "VTHC_FDCTHCLEVentZStaSet7_enum"
  VTHC_FDCTHCLEVentZStaSet7_enum_Inproc/1 -> UnitConverter827/1
  UnitConverter827/1 -> VOUTP_FDCTHCLEVentZStaSet7_enum/1  "VOUTP_FDCTHCLEVentZStaSet7_enum"
  VTHC_FDCTHCCLEVentZStaSet1_enum/1 -> VTHC_FDCTHCCLEVentZStaSet1_enum_Inproc/1  "VTHC_FDCTHCCLEVentZStaSet1_enum"
  VTHC_FDCTHCCLEVentZStaSet1_enum_Inproc/1 -> UnitConverter828/1
  UnitConverter828/1 -> VOUTP_FDCTHCCLEVentZStaSet1_enum/1  "VOUTP_FDCTHCCLEVentZStaSet1_enum"
  VTHC_FDCTHCCLEVentZStaSet2_enum/1 -> VTHC_FDCTHCCLEVentZStaSet2_enum_Inproc/1  "VTHC_FDCTHCCLEVentZStaSet2_enum"
  VTHC_FDCTHCCLEVentZStaSet2_enum_Inproc/1 -> UnitConverter829/1
  UnitConverter829/1 -> VOUTP_FDCTHCCLEVentZStaSet2_enum/1  "VOUTP_FDCTHCCLEVentZStaSet2_enum"
  VTHC_FDCTHCCLEVentZStaSet3_enum/1 -> VTHC_FDCTHCCLEVentZStaSet3_enum_Inproc/1  "VTHC_FDCTHCCLEVentZStaSet3_enum"
  VTHC_FDCTHCCLEVentZStaSet3_enum_Inproc/1 -> UnitConverter830/1
  UnitConverter830/1 -> VOUTP_FDCTHCCLEVentZStaSet3_enum/1  "VOUTP_FDCTHCCLEVentZStaSet3_enum"
  VTHC_FDCTHCCLEVentZStaSet4_enum/1 -> VTHC_FDCTHCCLEVentZStaSet4_enum_Inproc/1  "VTHC_FDCTHCCLEVentZStaSet4_enum"
  VTHC_FDCTHCCLEVentZStaSet4_enum_Inproc/1 -> UnitConverter831/1
  UnitConverter831/1 -> VOUTP_FDCTHCCLEVentZStaSet4_enum/1  "VOUTP_FDCTHCCLEVentZStaSet4_enum"
  VTHC_FDCTHCCLEVentZStaSet5_enum/1 -> VTHC_FDCTHCCLEVentZStaSet5_enum_Inproc/1  "VTHC_FDCTHCCLEVentZStaSet5_enum"
  VTHC_FDCTHCCLEVentZStaSet5_enum_Inproc/1 -> UnitConverter832/1
  UnitConverter832/1 -> VOUTP_FDCTHCCLEVentZStaSet5_enum/1  "VOUTP_FDCTHCCLEVentZStaSet5_enum"
  VTHC_FDCTHCCLEVentZStaSet7_enum/1 -> VTHC_FDCTHCCLEVentZStaSet7_enum_Inproc/1  "VTHC_FDCTHCCLEVentZStaSet7_enum"
  VTHC_FDCTHCCLEVentZStaSet7_enum_Inproc/1 -> UnitConverter833/1
  UnitConverter833/1 -> VOUTP_FDCTHCCLEVentZStaSet7_enum/1  "VOUTP_FDCTHCCLEVentZStaSet7_enum"
  VTHC_FDCTHCREVentZStaSet1_enum/1 -> VTHC_FDCTHCREVentZStaSet1_enum_Inproc/1  "VTHC_FDCTHCREVentZStaSet1_enum"
  VTHC_FDCTHCREVentZStaSet1_enum_Inproc/1 -> UnitConverter834/1
  UnitConverter834/1 -> VOUTP_FDCTHCREVentZStaSet1_enum/1  "VOUTP_FDCTHCREVentZStaSet1_enum"
  VTHC_FDCTHCREVentZStaSet2_enum/1 -> VTHC_FDCTHCREVentZStaSet2_enum_Inproc/1  "VTHC_FDCTHCREVentZStaSet2_enum"
  VTHC_FDCTHCREVentZStaSet2_enum_Inproc/1 -> UnitConverter835/1
  UnitConverter835/1 -> VOUTP_FDCTHCREVentZStaSet2_enum/1  "VOUTP_FDCTHCREVentZStaSet2_enum"
  VTHC_FDCTHCREVentZStaSet3_enum/1 -> VTHC_FDCTHCREVentZStaSet3_enum_Inproc/1  "VTHC_FDCTHCREVentZStaSet3_enum"
  VTHC_FDCTHCREVentZStaSet3_enum_Inproc/1 -> UnitConverter836/1
  UnitConverter836/1 -> VOUTP_FDCTHCREVentZStaSet3_enum/1  "VOUTP_FDCTHCREVentZStaSet3_enum"
  VTHC_FDCTHCREVentZStaSet4_enum/1 -> VTHC_FDCTHCREVentZStaSet4_enum_Inproc/1  "VTHC_FDCTHCREVentZStaSet4_enum"
  VTHC_FDCTHCREVentZStaSet4_enum_Inproc/1 -> UnitConverter837/1
  UnitConverter837/1 -> VOUTP_FDCTHCREVentZStaSet4_enum/1  "VOUTP_FDCTHCREVentZStaSet4_enum"
  VTHC_FDCTHCREVentZStaSet5_enum/1 -> VTHC_FDCTHCREVentZStaSet5_enum_Inproc/1  "VTHC_FDCTHCREVentZStaSet5_enum"
  VTHC_FDCTHCREVentZStaSet5_enum_Inproc/1 -> UnitConverter838/1
  UnitConverter838/1 -> VOUTP_FDCTHCREVentZStaSet5_enum/1  "VOUTP_FDCTHCREVentZStaSet5_enum"
  VTHC_FDCTHCREVentZStaSet7_enum/1 -> VTHC_FDCTHCREVentZStaSet7_enum_Inproc/1  "VTHC_FDCTHCREVentZStaSet7_enum"
  VTHC_FDCTHCREVentZStaSet7_enum_Inproc/1 -> UnitConverter839/1
  UnitConverter839/1 -> VOUTP_FDCTHCREVentZStaSet7_enum/1  "VOUTP_FDCTHCREVentZStaSet7_enum"
  VTHC_FDCTHCCREVentZStaSet1_enum/1 -> VTHC_FDCTHCCREVentZStaSet1_enum_Inproc/1  "VTHC_FDCTHCCREVentZStaSet1_enum"
  VTHC_FDCTHCCREVentZStaSet1_enum_Inproc/1 -> UnitConverter840/1
  UnitConverter840/1 -> VOUTP_FDCTHCCREVentZStaSet1_enum/1  "VOUTP_FDCTHCCREVentZStaSet1_enum"
  VTHC_FDCTHCCREVentZStaSet2_enum/1 -> VTHC_FDCTHCCREVentZStaSet2_enum_Inproc/1  "VTHC_FDCTHCCREVentZStaSet2_enum"
  VTHC_FDCTHCCREVentZStaSet2_enum_Inproc/1 -> UnitConverter841/1
  UnitConverter841/1 -> VOUTP_FDCTHCCREVentZStaSet2_enum/1  "VOUTP_FDCTHCCREVentZStaSet2_enum"
  VTHC_FDCTHCCREVentZStaSet3_enum/1 -> VTHC_FDCTHCCREVentZStaSet3_enum_Inproc/1  "VTHC_FDCTHCCREVentZStaSet3_enum"
  VTHC_FDCTHCCREVentZStaSet3_enum_Inproc/1 -> UnitConverter842/1
  UnitConverter842/1 -> VOUTP_FDCTHCCREVentZStaSet3_enum/1  "VOUTP_FDCTHCCREVentZStaSet3_enum"
  VTHC_FDCTHCCREVentZStaSet4_enum/1 -> VTHC_FDCTHCCREVentZStaSet4_enum_Inproc/1  "VTHC_FDCTHCCREVentZStaSet4_enum"
  VTHC_FDCTHCCREVentZStaSet4_enum_Inproc/1 -> UnitConverter843/1
  UnitConverter843/1 -> VOUTP_FDCTHCCREVentZStaSet4_enum/1  "VOUTP_FDCTHCCREVentZStaSet4_enum"
  VTHC_FDCTHCCREVentZStaSet5_enum/1 -> VTHC_FDCTHCCREVentZStaSet5_enum_Inproc/1  "VTHC_FDCTHCCREVentZStaSet5_enum"
  VTHC_FDCTHCCREVentZStaSet5_enum_Inproc/1 -> UnitConverter844/1
  UnitConverter844/1 -> VOUTP_FDCTHCCREVentZStaSet5_enum/1  "VOUTP_FDCTHCCREVentZStaSet5_enum"
  VTHC_FDCTHCCREVentZStaSet7_enum/1 -> VTHC_FDCTHCCREVentZStaSet7_enum_Inproc/1  "VTHC_FDCTHCCREVentZStaSet7_enum"
  VTHC_FDCTHCCREVentZStaSet7_enum_Inproc/1 -> UnitConverter845/1
  UnitConverter845/1 -> VOUTP_FDCTHCCREVentZStaSet7_enum/1  "VOUTP_FDCTHCCREVentZStaSet7_enum"
  VTHC_FDCTHCLEVentYStaSet1_enum/1 -> VTHC_FDCTHCLEVentYStaSet1_enum_Inproc/1  "VTHC_FDCTHCLEVentYStaSet1_enum"
  VTHC_FDCTHCLEVentYStaSet1_enum_Inproc/1 -> UnitConverter846/1
  UnitConverter846/1 -> VOUTP_FDCTHCLEVentYStaSet1_enum/1  "VOUTP_FDCTHCLEVentYStaSet1_enum"
  VTHC_FDCTHCLEVentYStaSet2_enum/1 -> VTHC_FDCTHCLEVentYStaSet2_enum_Inproc/1  "VTHC_FDCTHCLEVentYStaSet2_enum"
  VTHC_FDCTHCLEVentYStaSet2_enum_Inproc/1 -> UnitConverter847/1
  UnitConverter847/1 -> VOUTP_FDCTHCLEVentYStaSet2_enum/1  "VOUTP_FDCTHCLEVentYStaSet2_enum"
  VTHC_FDCTHCLEVentYStaSet3_enum/1 -> VTHC_FDCTHCLEVentYStaSet3_enum_Inproc/1  "VTHC_FDCTHCLEVentYStaSet3_enum"
  VTHC_FDCTHCLEVentYStaSet3_enum_Inproc/1 -> UnitConverter848/1
  UnitConverter848/1 -> VOUTP_FDCTHCLEVentYStaSet3_enum/1  "VOUTP_FDCTHCLEVentYStaSet3_enum"
  VTHC_FDCTHCLEVentYStaSet4_enum/1 -> VTHC_FDCTHCLEVentYStaSet4_enum_Inproc/1  "VTHC_FDCTHCLEVentYStaSet4_enum"
  VTHC_FDCTHCLEVentYStaSet4_enum_Inproc/1 -> UnitConverter849/1
  UnitConverter849/1 -> VOUTP_FDCTHCLEVentYStaSet4_enum/1  "VOUTP_FDCTHCLEVentYStaSet4_enum"
  VTHC_FDCTHCLEVentYStaSet5_enum/1 -> VTHC_FDCTHCLEVentYStaSet5_enum_Inproc/1  "VTHC_FDCTHCLEVentYStaSet5_enum"
  VTHC_FDCTHCLEVentYStaSet5_enum_Inproc/1 -> UnitConverter850/1
  UnitConverter850/1 -> VOUTP_FDCTHCLEVentYStaSet5_enum/1  "VOUTP_FDCTHCLEVentYStaSet5_enum"
  VTHC_FDCTHCLEVentYStaSet7_enum/1 -> VTHC_FDCTHCLEVentYStaSet7_enum_Inproc/1  "VTHC_FDCTHCLEVentYStaSet7_enum"
  VTHC_FDCTHCLEVentYStaSet7_enum_Inproc/1 -> UnitConverter851/1
  UnitConverter851/1 -> VOUTP_FDCTHCLEVentYStaSet7_enum/1  "VOUTP_FDCTHCLEVentYStaSet7_enum"
  VTHC_FDCTHCCLEVentYStaSet1_enum/1 -> VTHC_FDCTHCCLEVentYStaSet1_enum_Inproc/1  "VTHC_FDCTHCCLEVentYStaSet1_enum"
  VTHC_FDCTHCCLEVentYStaSet1_enum_Inproc/1 -> UnitConverter852/1
  UnitConverter852/1 -> VOUTP_FDCTHCCLEVentYStaSet1_enum/1  "VOUTP_FDCTHCCLEVentYStaSet1_enum"
  VTHC_FDCTHCCLEVentYStaSet2_enum/1 -> VTHC_FDCTHCCLEVentYStaSet2_enum_Inproc/1  "VTHC_FDCTHCCLEVentYStaSet2_enum"
  VTHC_FDCTHCCLEVentYStaSet2_enum_Inproc/1 -> UnitConverter853/1
  UnitConverter853/1 -> VOUTP_FDCTHCCLEVentYStaSet2_enum/1  "VOUTP_FDCTHCCLEVentYStaSet2_enum"
  VTHC_FDCTHCCLEVentYStaSet3_enum/1 -> VTHC_FDCTHCCLEVentYStaSet3_enum_Inproc/1  "VTHC_FDCTHCCLEVentYStaSet3_enum"
  VTHC_FDCTHCCLEVentYStaSet3_enum_Inproc/1 -> UnitConverter854/1
  UnitConverter854/1 -> VOUTP_FDCTHCCLEVentYStaSet3_enum/1  "VOUTP_FDCTHCCLEVentYStaSet3_enum"
  VTHC_FDCTHCCLEVentYStaSet4_enum/1 -> VTHC_FDCTHCCLEVentYStaSet4_enum_Inproc/1  "VTHC_FDCTHCCLEVentYStaSet4_enum"
  VTHC_FDCTHCCLEVentYStaSet4_enum_Inproc/1 -> UnitConverter855/1
  UnitConverter855/1 -> VOUTP_FDCTHCCLEVentYStaSet4_enum/1  "VOUTP_FDCTHCCLEVentYStaSet4_enum"
  VTHC_FDCTHCCLEVentYStaSet5_enum/1 -> VTHC_FDCTHCCLEVentYStaSet5_enum_Inproc/1  "VTHC_FDCTHCCLEVentYStaSet5_enum"
  VTHC_FDCTHCCLEVentYStaSet5_enum_Inproc/1 -> UnitConverter856/1
  UnitConverter856/1 -> VOUTP_FDCTHCCLEVentYStaSet5_enum/1  "VOUTP_FDCTHCCLEVentYStaSet5_enum"
  VTHC_FDCTHCCLEVentYStaSet7_enum/1 -> VTHC_FDCTHCCLEVentYStaSet7_enum_Inproc/1  "VTHC_FDCTHCCLEVentYStaSet7_enum"
  VTHC_FDCTHCCLEVentYStaSet7_enum_Inproc/1 -> UnitConverter857/1
  UnitConverter857/1 -> VOUTP_FDCTHCCLEVentYStaSet7_enum/1  "VOUTP_FDCTHCCLEVentYStaSet7_enum"
  VTHC_FDCTHCREVentYStaSet1_enum/1 -> VTHC_FDCTHCREVentYStaSet1_enum_Inproc/1  "VTHC_FDCTHCREVentYStaSet1_enum"
  VTHC_FDCTHCREVentYStaSet1_enum_Inproc/1 -> UnitConverter858/1
  UnitConverter858/1 -> VOUTP_FDCTHCREVentYStaSet1_enum/1  "VOUTP_FDCTHCREVentYStaSet1_enum"
  VTHC_FDCTHCREVentYStaSet2_enum/1 -> VTHC_FDCTHCREVentYStaSet2_enum_Inproc/1  "VTHC_FDCTHCREVentYStaSet2_enum"
  VTHC_FDCTHCREVentYStaSet2_enum_Inproc/1 -> UnitConverter859/1
  UnitConverter859/1 -> VOUTP_FDCTHCREVentYStaSet2_enum/1  "VOUTP_FDCTHCREVentYStaSet2_enum"
  VTHC_FDCTHCREVentYStaSet3_enum/1 -> VTHC_FDCTHCREVentYStaSet3_enum_Inproc/1  "VTHC_FDCTHCREVentYStaSet3_enum"
  VTHC_FDCTHCREVentYStaSet3_enum_Inproc/1 -> UnitConverter860/1
  UnitConverter860/1 -> VOUTP_FDCTHCREVentYStaSet3_enum/1  "VOUTP_FDCTHCREVentYStaSet3_enum"
  VTHC_FDCTHCREVentYStaSet4_enum/1 -> VTHC_FDCTHCREVentYStaSet4_enum_Inproc/1  "VTHC_FDCTHCREVentYStaSet4_enum"
  VTHC_FDCTHCREVentYStaSet4_enum_Inproc/1 -> UnitConverter861/1
  UnitConverter861/1 -> VOUTP_FDCTHCREVentYStaSet4_enum/1  "VOUTP_FDCTHCREVentYStaSet4_enum"
  VTHC_FDCTHCREVentYStaSet5_enum/1 -> VTHC_FDCTHCREVentYStaSet5_enum_Inproc/1  "VTHC_FDCTHCREVentYStaSet5_enum"
  VTHC_FDCTHCREVentYStaSet5_enum_Inproc/1 -> UnitConverter862/1
  UnitConverter862/1 -> VOUTP_FDCTHCREVentYStaSet5_enum/1  "VOUTP_FDCTHCREVentYStaSet5_enum"
  VTHC_FDCTHCREVentYStaSet7_enum/1 -> VTHC_FDCTHCREVentYStaSet7_enum_Inproc/1  "VTHC_FDCTHCREVentYStaSet7_enum"
  VTHC_FDCTHCREVentYStaSet7_enum_Inproc/1 -> UnitConverter863/1
  UnitConverter863/1 -> VOUTP_FDCTHCREVentYStaSet7_enum/1  "VOUTP_FDCTHCREVentYStaSet7_enum"
  VTHC_FDCTHCCREVentYStaSet1_enum/1 -> VTHC_FDCTHCCREVentYStaSet1_enum_Inproc/1  "VTHC_FDCTHCCREVentYStaSet1_enum"
  VTHC_FDCTHCCREVentYStaSet1_enum_Inproc/1 -> UnitConverter864/1
  UnitConverter864/1 -> VOUTP_FDCTHCCREVentYStaSet1_enum/1  "VOUTP_FDCTHCCREVentYStaSet1_enum"
  VTHC_FDCTHCCREVentYStaSet2_enum/1 -> VTHC_FDCTHCCREVentYStaSet2_enum_Inproc/1  "VTHC_FDCTHCCREVentYStaSet2_enum"
  VTHC_FDCTHCCREVentYStaSet2_enum_Inproc/1 -> UnitConverter865/1
  UnitConverter865/1 -> VOUTP_FDCTHCCREVentYStaSet2_enum/1  "VOUTP_FDCTHCCREVentYStaSet2_enum"
  VTHC_FDCTHCCREVentYStaSet3_enum/1 -> VTHC_FDCTHCCREVentYStaSet3_enum_Inproc/1  "VTHC_FDCTHCCREVentYStaSet3_enum"
  VTHC_FDCTHCCREVentYStaSet3_enum_Inproc/1 -> UnitConverter866/1
  UnitConverter866/1 -> VOUTP_FDCTHCCREVentYStaSet3_enum/1  "VOUTP_FDCTHCCREVentYStaSet3_enum"
  VTHC_FDCTHCCREVentYStaSet4_enum/1 -> VTHC_FDCTHCCREVentYStaSet4_enum_Inproc/1  "VTHC_FDCTHCCREVentYStaSet4_enum"
  VTHC_FDCTHCCREVentYStaSet4_enum_Inproc/1 -> UnitConverter867/1
  UnitConverter867/1 -> VOUTP_FDCTHCCREVentYStaSet4_enum/1  "VOUTP_FDCTHCCREVentYStaSet4_enum"
  VTHC_FDCTHCCREVentYStaSet5_enum/1 -> VTHC_FDCTHCCREVentYStaSet5_enum_Inproc/1  "VTHC_FDCTHCCREVentYStaSet5_enum"
  VTHC_FDCTHCCREVentYStaSet5_enum_Inproc/1 -> UnitConverter868/1
  UnitConverter868/1 -> VOUTP_FDCTHCCREVentYStaSet5_enum/1  "VOUTP_FDCTHCCREVentYStaSet5_enum"
  VTHC_FDCTHCCREVentYStaSet7_enum/1 -> VTHC_FDCTHCCREVentYStaSet7_enum_Inproc/1  "VTHC_FDCTHCCREVentYStaSet7_enum"
  VTHC_FDCTHCCREVentYStaSet7_enum_Inproc/1 -> UnitConverter869/1
  UnitConverter869/1 -> VOUTP_FDCTHCCREVentYStaSet7_enum/1  "VOUTP_FDCTHCCREVentYStaSet7_enum"
  VTHC_SettempZon1Set1_enum/1 -> VTHC_SettempZon1Set1_enum_Inproc/1  "VTHC_SettempZon1Set1_enum"
  VTHC_SettempZon1Set1_enum_Inproc/1 -> UnitConverter870/1
  UnitConverter870/1 -> VOUTP_SettempZon1Set1_enum/1  "VOUTP_SettempZon1Set1_enum"
  VTHC_SettempZon1Set2_enum/1 -> VTHC_SettempZon1Set2_enum_Inproc/1  "VTHC_SettempZon1Set2_enum"
  VTHC_SettempZon1Set2_enum_Inproc/1 -> UnitConverter871/1
  UnitConverter871/1 -> VOUTP_SettempZon1Set2_enum/1  "VOUTP_SettempZon1Set2_enum"
  VTHC_SettempZon1Set3_enum/1 -> VTHC_SettempZon1Set3_enum_Inproc/1  "VTHC_SettempZon1Set3_enum"
  VTHC_SettempZon1Set3_enum_Inproc/1 -> UnitConverter872/1
  UnitConverter872/1 -> VOUTP_SettempZon1Set3_enum/1  "VOUTP_SettempZon1Set3_enum"
  VTHC_SettempZon1Set4_enum/1 -> VTHC_SettempZon1Set4_enum_Inproc/1  "VTHC_SettempZon1Set4_enum"
  VTHC_SettempZon1Set4_enum_Inproc/1 -> UnitConverter873/1
  UnitConverter873/1 -> VOUTP_SettempZon1Set4_enum/1  "VOUTP_SettempZon1Set4_enum"
  VTHC_SettempZon1Set5_enum/1 -> VTHC_SettempZon1Set5_enum_Inproc/1  "VTHC_SettempZon1Set5_enum"
  VTHC_SettempZon1Set5_enum_Inproc/1 -> UnitConverter874/1
  UnitConverter874/1 -> VOUTP_SettempZon1Set5_enum/1  "VOUTP_SettempZon1Set5_enum"
  VTHC_SettempZon1Set7_enum/1 -> VTHC_SettempZon1Set7_enum_Inproc/1  "VTHC_SettempZon1Set7_enum"
  VTHC_SettempZon1Set7_enum_Inproc/1 -> UnitConverter875/1
  UnitConverter875/1 -> VOUTP_SettempZon1Set7_enum/1  "VOUTP_SettempZon1Set7_enum"
  VTHC_ACModeSet123_enum/1 -> VTHC_ACModeSet123_enum_Inproc/1  "VTHC_ACModeSet123_enum"
  VTHC_ACModeSet123_enum_Inproc/1 -> UnitConverter876/1
  UnitConverter876/1 -> VOUTP_ACModeSet123_enum/1  "VOUTP_ACModeSet123_enum"
  VTHC_ACModeSet457_enum/1 -> VTHC_ACModeSet457_enum_Inproc/1  "VTHC_ACModeSet457_enum"
  VTHC_ACModeSet457_enum_Inproc/1 -> UnitConverter877/1
  UnitConverter877/1 -> VOUTP_ACModeSet457_enum/1  "VOUTP_ACModeSet457_enum"
  VTHC_FACESet_enum/1 -> VTHC_FACESet_enum_Inproc/1  "VTHC_FACESet_enum"
  VTHC_FACESet_enum_Inproc/1 -> UnitConverter878/1
  UnitConverter878/1 -> VOUTP_FACESet_enum/1  "VOUTP_FACESet_enum"
  VTHC_FOOTSet_enum/1 -> VTHC_FOOTSet_enum_Inproc/1  "VTHC_FOOTSet_enum"
  VTHC_FOOTSet_enum_Inproc/1 -> UnitConverter879/1
  UnitConverter879/1 -> VOUTP_FOOTSet_enum/1  "VOUTP_FOOTSet_enum"
  VTHC_FrostSet_enum/1 -> VTHC_FrostSet_enum_Inproc/1  "VTHC_FrostSet_enum"
  VTHC_FrostSet_enum_Inproc/1 -> UnitConverter880/1
  UnitConverter880/1 -> VOUTP_FrostSet_enum/1  "VOUTP_FrostSet_enum"
  VTHC_LVentEN_flg/1 -> VTHC_LVentEN_flg_Inproc/1  "VTHC_LVentEN_flg"
  VTHC_LVentEN_flg_Inproc/1 -> UnitConverter881/1
  UnitConverter881/1 -> VOUTP_LVentEN_flg/1  "VOUTP_LVentEN_flg"
  VTHC_CLVentEN_flg/1 -> VTHC_CLVentEN_flg_Inproc/1  "VTHC_CLVentEN_flg"
  VTHC_CLVentEN_flg_Inproc/1 -> UnitConverter882/1
  UnitConverter882/1 -> VOUTP_CLVentEN_flg/1  "VOUTP_CLVentEN_flg"
  VTHC_RVentEN_flg/1 -> VTHC_RVentEN_flg_Inproc/1  "VTHC_RVentEN_flg"
  VTHC_RVentEN_flg_Inproc/1 -> UnitConverter883/1
  UnitConverter883/1 -> VOUTP_RVentEN_flg/1  "VOUTP_RVentEN_flg"
  VTHC_CRVentEN_flg/1 -> VTHC_CRVentEN_flg_Inproc/1  "VTHC_CRVentEN_flg"
  VTHC_CRVentEN_flg_Inproc/1 -> UnitConverter884/1
  UnitConverter884/1 -> VOUTP_CRVentEN_flg/1  "VOUTP_CRVentEN_flg"
  VTHC_FDCFGSLearnCmd_enum/1 -> VTHC_FDCFGSLearnCmd_enum_Inproc/1  "VTHC_FDCFGSLearnCmd_enum"
  VTHC_FDCFGSLearnCmd_enum_Inproc/1 -> UnitConverter885/1
  UnitConverter885/1 -> VOUTP_FDCFGSLearnCmd_enum/1  "VOUTP_FDCFGSLearnCmd_enum"
  VTHC_FDCFGSFuncSta_flg/1 -> VTHC_FDCFGSFuncSta_flg_Inproc/1  "VTHC_FDCFGSFuncSta_flg"
  VTHC_FDCFGSFuncSta_flg_Inproc/1 -> UnitConverter886/1
  UnitConverter886/1 -> VOUTP_FDCFGSFuncSta_flg/1  "VOUTP_FDCFGSFuncSta_flg"
  VTHC_THSysErrlampReq_flg/1 -> VTHC_THSysErrlampReq_flg_Inproc/1  "VTHC_THSysErrlampReq_flg"
  VTHC_THSysErrlampReq_flg_Inproc/1 -> UnitConverter887/1
  UnitConverter887/1 -> VOUTP_THSysErrlampReq_flg/1  "VOUTP_THSysErrlampReq_flg"
  VTPM_LFBatWarn_flg/1 -> VTPM_LFBatWarn_flg_Inproc/1  "VTPM_LFBatWarn_flg"
  VTPM_LFBatWarn_flg_Inproc/1 -> UnitConverter888/1
  UnitConverter888/1 -> VOUTP_LFBatWarn_flg/1  "VOUTP_LFBatWarn_flg"
  VTPM_RFBatWarn_flg/1 -> VTPM_RFBatWarn_flg_Inproc/1  "VTPM_RFBatWarn_flg"
  VTPM_RFBatWarn_flg_Inproc/1 -> UnitConverter889/1
  UnitConverter889/1 -> VOUTP_RFBatWarn_flg/1  "VOUTP_RFBatWarn_flg"
  VTPM_LRBatWarn_flg/1 -> VTPM_LRBatWarn_flg_Inproc/1  "VTPM_LRBatWarn_flg"
  VTPM_LRBatWarn_flg_Inproc/1 -> UnitConverter890/1
  UnitConverter890/1 -> VOUTP_LRBatWarn_flg/1  "VOUTP_LRBatWarn_flg"
  VTPM_RRBatWarn_flg/1 -> VTPM_RRBatWarn_flg_Inproc/1  "VTPM_RRBatWarn_flg"
  VTPM_RRBatWarn_flg_Inproc/1 -> UnitConverter891/1
  UnitConverter891/1 -> VOUTP_RRBatWarn_flg/1  "VOUTP_RRBatWarn_flg"
  VTPM_LFWheelPress_raw8/1 -> VTPM_LFWheelPress_raw8_Inproc/1  "VTPM_LFWheelPress_raw8"
  VTPM_LFWheelPress_raw8_Inproc/1 -> UnitConverter892/1
  UnitConverter892/1 -> VOUTP_LFWheelPress_raw8/1  "VOUTP_LFWheelPress_raw8"
  VTPM_RFWheelPress_raw8/1 -> VTPM_RFWheelPress_raw8_Inproc/1  "VTPM_RFWheelPress_raw8"
  VTPM_RFWheelPress_raw8_Inproc/1 -> UnitConverter893/1
  UnitConverter893/1 -> VOUTP_RFWheelPress_raw8/1  "VOUTP_RFWheelPress_raw8"
  VTPM_LRWheelPress_raw8/1 -> VTPM_LRWheelPress_raw8_Inproc/1  "VTPM_LRWheelPress_raw8"
  VTPM_LRWheelPress_raw8_Inproc/1 -> UnitConverter894/1
  UnitConverter894/1 -> VOUTP_LRWheelPress_raw8/1  "VOUTP_LRWheelPress_raw8"
  VTPM_RRWheelPress_raw8/1 -> VTPM_RRWheelPress_raw8_Inproc/1  "VTPM_RRWheelPress_raw8"
  VTPM_RRWheelPress_raw8_Inproc/1 -> UnitConverter895/1
  UnitConverter895/1 -> VOUTP_RRWheelPress_raw8/1  "VOUTP_RRWheelPress_raw8"
  VTPM_LFWheelTemp_C/1 -> VTPM_LFWheelTemp_C_Inproc/1  "VTPM_LFWheelTemp_C"
  VTPM_LFWheelTemp_C_Inproc/1 -> UnitConverter896/1
  UnitConverter896/1 -> VOUTP_LFWheelTemp_C/1  "VOUTP_LFWheelTemp_C"
  VTPM_RFWheelTemp_C/1 -> VTPM_RFWheelTemp_C_Inproc/1  "VTPM_RFWheelTemp_C"
  VTPM_RFWheelTemp_C_Inproc/1 -> UnitConverter897/1
  UnitConverter897/1 -> VOUTP_RFWheelTemp_C/1  "VOUTP_RFWheelTemp_C"
  VTPM_LRWheelTemp_C/1 -> VTPM_LRWheelTemp_C_Inproc/1  "VTPM_LRWheelTemp_C"
  VTPM_LRWheelTemp_C_Inproc/1 -> UnitConverter898/1
  UnitConverter898/1 -> VOUTP_LRWheelTemp_C/1  "VOUTP_LRWheelTemp_C"
  VTPM_RRWheelTemp_C/1 -> VTPM_RRWheelTemp_C_Inproc/1  "VTPM_RRWheelTemp_C"
  VTPM_RRWheelTemp_C_Inproc/1 -> UnitConverter899/1
  UnitConverter899/1 -> VOUTP_RRWheelTemp_C/1  "VOUTP_RRWheelTemp_C"
  VTPM_LFSensorFail_flg/1 -> VTPM_LFSensorFail_flg_Inproc/1  "VTPM_LFSensorFail_flg"
  VTPM_LFSensorFail_flg_Inproc/1 -> UnitConverter900/1
  UnitConverter900/1 -> VOUTP_LFSensorFail_flg/1  "VOUTP_LFSensorFail_flg"
  VTPM_RFSensorFail_flg/1 -> VTPM_RFSensorFail_flg_Inproc/1  "VTPM_RFSensorFail_flg"
  VTPM_RFSensorFail_flg_Inproc/1 -> UnitConverter901/1
  UnitConverter901/1 -> VOUTP_RFSensorFail_flg/1  "VOUTP_RFSensorFail_flg"
  VTPM_LRSensorFail_flg/1 -> VTPM_LRSensorFail_flg_Inproc/1  "VTPM_LRSensorFail_flg"
  VTPM_LRSensorFail_flg_Inproc/1 -> UnitConverter902/1
  UnitConverter902/1 -> VOUTP_LRSensorFail_flg/1  "VOUTP_LRSensorFail_flg"
  VTPM_RRSensorFail_flg/1 -> VTPM_RRSensorFail_flg_Inproc/1  "VTPM_RRSensorFail_flg"
  VTPM_RRSensorFail_flg_Inproc/1 -> UnitConverter903/1
  UnitConverter903/1 -> VOUTP_RRSensorFail_flg/1  "VOUTP_RRSensorFail_flg"
  VTPM_LFWheelDebug_flg/1 -> VTPM_LFWheelDebug_flg_Inproc/1  "VTPM_LFWheelDebug_flg"
  VTPM_LFWheelDebug_flg_Inproc/1 -> UnitConverter904/1
  UnitConverter904/1 -> VOUTP_LFWheelDebug_flg/1  "VOUTP_LFWheelDebug_flg"
  VTPM_LRWheelDebug_flg/1 -> VTPM_LRWheelDebug_flg_Inproc/1  "VTPM_LRWheelDebug_flg"
  VTPM_LRWheelDebug_flg_Inproc/1 -> UnitConverter905/1
  UnitConverter905/1 -> VOUTP_LRWheelDebug_flg/1  "VOUTP_LRWheelDebug_flg"
  VTPM_RFWheelDebug_flg/1 -> VTPM_RFWheelDebug_flg_Inproc/1  "VTPM_RFWheelDebug_flg"
  VTPM_RFWheelDebug_flg_Inproc/1 -> UnitConverter906/1
  UnitConverter906/1 -> VOUTP_RFWheelDebug_flg/1  "VOUTP_RFWheelDebug_flg"
  VTPM_RRWheelDebug_flg/1 -> VTPM_RRWheelDebug_flg_Inproc/1  "VTPM_RRWheelDebug_flg"
  VTPM_RRWheelDebug_flg_Inproc/1 -> UnitConverter907/1
  UnitConverter907/1 -> VOUTP_RRWheelDebug_flg/1  "VOUTP_RRWheelDebug_flg"
  VTPM_TPMSResButtAllow_flg/1 -> VTPM_TPMSResButtAllow_flg_Inproc/1  "VTPM_TPMSResButtAllow_flg"
  VTPM_TPMSResButtAllow_flg_Inproc/1 -> UnitConverter908/1
  UnitConverter908/1 -> VOUTP_TPMSResButtAllow_flg/1  "VOUTP_TPMSResButtAllow_flg"
  VTPM_TPMSCaliButtAllow_flg/1 -> VTPM_TPMSCaliButtAllow_flg_Inproc/1  "VTPM_TPMSCaliButtAllow_flg"
  VTPM_TPMSCaliButtAllow_flg_Inproc/1 -> UnitConverter909/1
  UnitConverter909/1 -> VOUTP_TPMSCaliButtAllow_flg/1  "VOUTP_TPMSCaliButtAllow_flg"
  VTPM_LFPressIndi_enum/1 -> VTPM_LFPressIndi_enum_Inproc/1  "VTPM_LFPressIndi_enum"
  VTPM_LFPressIndi_enum_Inproc/1 -> UnitConverter910/1
  UnitConverter910/1 -> VOUTP_LFPressIndi_enum/1  "VOUTP_LFPressIndi_enum"
  VTPM_RFPressIndi_enum/1 -> VTPM_RFPressIndi_enum_Inproc/1  "VTPM_RFPressIndi_enum"
  VTPM_RFPressIndi_enum_Inproc/1 -> UnitConverter911/1
  UnitConverter911/1 -> VOUTP_RFPressIndi_enum/1  "VOUTP_RFPressIndi_enum"
  VTPM_LRPressIndi_enum/1 -> VTPM_LRPressIndi_enum_Inproc/1  "VTPM_LRPressIndi_enum"
  VTPM_LRPressIndi_enum_Inproc/1 -> UnitConverter912/1
  UnitConverter912/1 -> VOUTP_LRPressIndi_enum/1  "VOUTP_LRPressIndi_enum"
  VTPM_RRPressIndi_enum/1 -> VTPM_RRPressIndi_enum_Inproc/1  "VTPM_RRPressIndi_enum"
  VTPM_RRPressIndi_enum_Inproc/1 -> UnitConverter913/1
  UnitConverter913/1 -> VOUTP_RRPressIndi_enum/1  "VOUTP_RRPressIndi_enum"
  VTPM_TPMSWarnIndi_enum/1 -> VTPM_TPMSWarnIndi_enum_Inproc/1  "VTPM_TPMSWarnIndi_enum"
  VTPM_TPMSWarnIndi_enum_Inproc/1 -> UnitConverter914/1
  UnitConverter914/1 -> VOUTP_TPMSWarnIndi_enum/1  "VOUTP_TPMSWarnIndi_enum"
  VTPM_LFWheelTmpIndi_flg/1 -> VTPM_LFWheelTmpIndi_flg_Inproc/1  "VTPM_LFWheelTmpIndi_flg"
  VTPM_LFWheelTmpIndi_flg_Inproc/1 -> UnitConverter915/1
  UnitConverter915/1 -> VOUTP_LFWheelTmpIndi_flg/1  "VOUTP_LFWheelTmpIndi_flg"
  VTPM_RFWheelTmpIndi_flg/1 -> VTPM_RFWheelTmpIndi_flg_Inproc/1  "VTPM_RFWheelTmpIndi_flg"
  VTPM_RFWheelTmpIndi_flg_Inproc/1 -> UnitConverter916/1
  UnitConverter916/1 -> VOUTP_RFWheelTmpIndi_flg/1  "VOUTP_RFWheelTmpIndi_flg"
  VTPM_LRWheelTmpIndi_flg/1 -> VTPM_LRWheelTmpIndi_flg_Inproc/1  "VTPM_LRWheelTmpIndi_flg"
  VTPM_LRWheelTmpIndi_flg_Inproc/1 -> UnitConverter917/1
  UnitConverter917/1 -> VOUTP_LRWheelTmpIndi_flg/1  "VOUTP_LRWheelTmpIndi_flg"
  VTPM_RRWheelTmpIndi_flg/1 -> VTPM_RRWheelTmpIndi_flg_Inproc/1  "VTPM_RRWheelTmpIndi_flg"
  VTPM_RRWheelTmpIndi_flg_Inproc/1 -> UnitConverter918/1
  UnitConverter918/1 -> VOUTP_RRWheelTmpIndi_flg/1  "VOUTP_RRWheelTmpIndi_flg"
  VTPM_LFWheelPSW_raw8/1 -> VTPM_LFWheelPSW_raw8_Inproc/1  "VTPM_LFWheelPSW_raw8"
  VTPM_LFWheelPSW_raw8_Inproc/1 -> UnitConverter919/1
  UnitConverter919/1 -> VOUTP_LFWheelPSW_raw8/1  "VOUTP_LFWheelPSW_raw8"
  VTPM_LRWheelPSW_raw8/1 -> VTPM_LRWheelPSW_raw8_Inproc/1  "VTPM_LRWheelPSW_raw8"
  VTPM_LRWheelPSW_raw8_Inproc/1 -> UnitConverter920/1
  UnitConverter920/1 -> VOUTP_LRWheelPSW_raw8/1  "VOUTP_LRWheelPSW_raw8"
  VTPM_RFWheelPSW_raw8/1 -> VTPM_RFWheelPSW_raw8_Inproc/1  "VTPM_RFWheelPSW_raw8"
  VTPM_RFWheelPSW_raw8_Inproc/1 -> UnitConverter921/1
  UnitConverter921/1 -> VOUTP_RFWheelPSW_raw8/1  "VOUTP_RFWheelPSW_raw8"
  VTPM_RRWheelPSW_raw8/1 -> VTPM_RRWheelPSW_raw8_Inproc/1  "VTPM_RRWheelPSW_raw8"
  VTPM_RRWheelPSW_raw8_Inproc/1 -> UnitConverter922/1
  UnitConverter922/1 -> VOUTP_RRWheelPSW_raw8/1  "VOUTP_RRWheelPSW_raw8"
  VTPM_CWheelTips_enum/1 -> VTPM_CWheelTips_enum_Inproc/1  "VTPM_CWheelTips_enum"
  VTPM_CWheelTips_enum_Inproc/1 -> UnitConverter923/1
  UnitConverter923/1 -> VOUTP_CWheelTips_enum/1  "VOUTP_CWheelTips_enum"
  VTPM_AutoLTips_enum/1 -> VTPM_AutoLTips_enum_Inproc/1  "VTPM_AutoLTips_enum"
  VTPM_AutoLTips_enum_Inproc/1 -> UnitConverter924/1
  UnitConverter924/1 -> VOUTP_AutoLTips_enum/1  "VOUTP_AutoLTips_enum"
  VTPM_LFSensorMode_flg/1 -> VTPM_LFSensorMode_flg_Inproc/1  "VTPM_LFSensorMode_flg"
  VTPM_LFSensorMode_flg_Inproc/1 -> UnitConverter925/1
  UnitConverter925/1 -> VOUTP_LFSensorMode_flg/1  "VOUTP_LFSensorMode_flg"
  VTPM_RFSensorMode_flg/1 -> VTPM_RFSensorMode_flg_Inproc/1  "VTPM_RFSensorMode_flg"
  VTPM_RFSensorMode_flg_Inproc/1 -> UnitConverter926/1
  UnitConverter926/1 -> VOUTP_RFSensorMode_flg/1  "VOUTP_RFSensorMode_flg"
  VTPM_LRSensorMode_flg/1 -> VTPM_LRSensorMode_flg_Inproc/1  "VTPM_LRSensorMode_flg"
  VTPM_LRSensorMode_flg_Inproc/1 -> UnitConverter927/1
  UnitConverter927/1 -> VOUTP_LRSensorMode_flg/1  "VOUTP_LRSensorMode_flg"
  VTPM_RRSensorMode_flg/1 -> VTPM_RRSensorMode_flg_Inproc/1  "VTPM_RRSensorMode_flg"
  VTPM_RRSensorMode_flg_Inproc/1 -> UnitConverter928/1
  UnitConverter928/1 -> VOUTP_RRSensorMode_flg/1  "VOUTP_RRSensorMode_flg"
  VTPM_S1ID_raw32/1 -> VTPM_S1ID_raw32_Inproc/1  "VTPM_S1ID_raw32"
  VTPM_S1ID_raw32_Inproc/1 -> UnitConverter929/1
  UnitConverter929/1 -> VOUTP_S1ID_raw32/1  "VOUTP_S1ID_raw32"
  VTPM_S2ID_raw32/1 -> VTPM_S2ID_raw32_Inproc/1  "VTPM_S2ID_raw32"
  VTPM_S2ID_raw32_Inproc/1 -> UnitConverter930/1
  UnitConverter930/1 -> VOUTP_S2ID_raw32/1  "VOUTP_S2ID_raw32"
  VTPM_S3ID_raw32/1 -> VTPM_S3ID_raw32_Inproc/1  "VTPM_S3ID_raw32"
  VTPM_S3ID_raw32_Inproc/1 -> UnitConverter931/1
  UnitConverter931/1 -> VOUTP_S3ID_raw32/1  "VOUTP_S3ID_raw32"
  VTPM_S4ID_raw32/1 -> VTPM_S4ID_raw32_Inproc/1  "VTPM_S4ID_raw32"
  VTPM_S4ID_raw32_Inproc/1 -> UnitConverter932/1
  UnitConverter932/1 -> VOUTP_S4ID_raw32/1  "VOUTP_S4ID_raw32"
  VTPM_S1L_enum/1 -> VTPM_S1L_enum_Inproc/1  "VTPM_S1L_enum"
  VTPM_S1L_enum_Inproc/1 -> UnitConverter933/1
  UnitConverter933/1 -> VOUTP_S1L_enum/1  "VOUTP_S1L_enum"
  VTPM_S2L_enum/1 -> VTPM_S2L_enum_Inproc/1  "VTPM_S2L_enum"
  VTPM_S2L_enum_Inproc/1 -> UnitConverter934/1
  UnitConverter934/1 -> VOUTP_S2L_enum/1  "VOUTP_S2L_enum"
  VTPM_S3L_enum/1 -> VTPM_S3L_enum_Inproc/1  "VTPM_S3L_enum"
  VTPM_S3L_enum_Inproc/1 -> UnitConverter935/1
  UnitConverter935/1 -> VOUTP_S3L_enum/1  "VOUTP_S3L_enum"
  VTPM_S4L_enum/1 -> VTPM_S4L_enum_Inproc/1  "VTPM_S4L_enum"
  VTPM_S4L_enum_Inproc/1 -> UnitConverter936/1
  UnitConverter936/1 -> VOUTP_S4L_enum/1  "VOUTP_S4L_enum"
  VTPM_ALFin_flg/1 -> VTPM_ALFin_flg_Inproc/1  "VTPM_ALFin_flg"
  VTPM_ALFin_flg_Inproc/1 -> UnitConverter937/1
  UnitConverter937/1 -> VOUTP_ALFin_flg/1  "VOUTP_ALFin_flg"
  VTPM_LFP20_raw8/1 -> VTPM_LFP20_raw8_Inproc/1  "VTPM_LFP20_raw8"
  VTPM_LFP20_raw8_Inproc/1 -> UnitConverter938/1
  UnitConverter938/1 -> VOUTP_LFP20_raw8/1  "VOUTP_LFP20_raw8"
  VTPM_RFP20_raw8/1 -> VTPM_RFP20_raw8_Inproc/1  "VTPM_RFP20_raw8"
  VTPM_RFP20_raw8_Inproc/1 -> UnitConverter939/1
  UnitConverter939/1 -> VOUTP_RFP20_raw8/1  "VOUTP_RFP20_raw8"
  VTPM_LRP20_raw8/1 -> VTPM_LRP20_raw8_Inproc/1  "VTPM_LRP20_raw8"
  VTPM_LRP20_raw8_Inproc/1 -> UnitConverter940/1
  UnitConverter940/1 -> VOUTP_LRP20_raw8/1  "VOUTP_LRP20_raw8"
  VTPM_RRP20_raw8/1 -> VTPM_RRP20_raw8_Inproc/1  "VTPM_RRP20_raw8"
  VTPM_RRP20_raw8_Inproc/1 -> UnitConverter941/1
  UnitConverter941/1 -> VOUTP_RRP20_raw8/1  "VOUTP_RRP20_raw8"
  VTPM_FAT_flg/1 -> VTPM_FAT_flg_Inproc/1  "VTPM_FAT_flg"
  VTPM_FAT_flg_Inproc/1 -> UnitConverter942/1
  UnitConverter942/1 -> VOUTP_FAT_flg/1  "VOUTP_FAT_flg"
  VTPM_IDin_raw32/1 -> VTPM_IDin_raw32_Inproc/1  "VTPM_IDin_raw32"
  VTPM_IDin_raw32_Inproc/1 -> UnitConverter943/1
  UnitConverter943/1 -> VOUTP_IDin_raw32/1  "VOUTP_IDin_raw32"
  VTPM_S1WheelDebugALTU_pct/1 -> VTPM_S1WheelDebugALTU_pct_Inproc/1  "VTPM_S1WheelDebugALTU_pct"
  VTPM_S1WheelDebugALTU_pct_Inproc/1 -> UnitConverter944/1
  UnitConverter944/1 -> VOUTP_S1WheelDebugALTU_pct/1  "VOUTP_S1WheelDebugALTU_pct"
  VTPM_S2WheelDebugALTU_pct/1 -> VTPM_S2WheelDebugALTU_pct_Inproc/1  "VTPM_S2WheelDebugALTU_pct"
  VTPM_S2WheelDebugALTU_pct_Inproc/1 -> UnitConverter945/1
  UnitConverter945/1 -> VOUTP_S2WheelDebugALTU_pct/1  "VOUTP_S2WheelDebugALTU_pct"
  VTPM_S3WheelDebugALTU_pct/1 -> VTPM_S3WheelDebugALTU_pct_Inproc/1  "VTPM_S3WheelDebugALTU_pct"
  VTPM_S3WheelDebugALTU_pct_Inproc/1 -> UnitConverter946/1
  UnitConverter946/1 -> VOUTP_S3WheelDebugALTU_pct/1  "VOUTP_S3WheelDebugALTU_pct"
  VTPM_S4WheelDebugALTU_pct/1 -> VTPM_S4WheelDebugALTU_pct_Inproc/1  "VTPM_S4WheelDebugALTU_pct"
  VTPM_S4WheelDebugALTU_pct_Inproc/1 -> UnitConverter947/1
  UnitConverter947/1 -> VOUTP_S4WheelDebugALTU_pct/1  "VOUTP_S4WheelDebugALTU_pct"
  VTPM_ID1messageALTU_raw8/1 -> VTPM_ID1messageALTU_raw8_Inproc/1  "VTPM_ID1messageALTU_raw8"
  VTPM_ID1messageALTU_raw8_Inproc/1 -> UnitConverter948/1
  UnitConverter948/1 -> VOUTP_ID1messageALTU_raw8/1  "VOUTP_ID1messageALTU_raw8"
  VTPM_ID2messageALTU_raw8/1 -> VTPM_ID2messageALTU_raw8_Inproc/1  "VTPM_ID2messageALTU_raw8"
  VTPM_ID2messageALTU_raw8_Inproc/1 -> UnitConverter949/1
  UnitConverter949/1 -> VOUTP_ID2messageALTU_raw8/1  "VOUTP_ID2messageALTU_raw8"
  VTPM_ID3messageALTU_raw8/1 -> VTPM_ID3messageALTU_raw8_Inproc/1  "VTPM_ID3messageALTU_raw8"
  VTPM_ID3messageALTU_raw8_Inproc/1 -> UnitConverter950/1
  UnitConverter950/1 -> VOUTP_ID3messageALTU_raw8/1  "VOUTP_ID3messageALTU_raw8"
  VTPM_ID4messageALTU_raw8/1 -> VTPM_ID4messageALTU_raw8_Inproc/1  "VTPM_ID4messageALTU_raw8"
  VTPM_ID4messageALTU_raw8_Inproc/1 -> UnitConverter951/1
  UnitConverter951/1 -> VOUTP_ID4messageALTU_raw8/1  "VOUTP_ID4messageALTU_raw8"
  VTPM_Chkfin_flg/1 -> VTPM_Chkfin_flg_Inproc/1  "VTPM_Chkfin_flg"
  VTPM_Chkfin_flg_Inproc/1 -> UnitConverter952/1
  UnitConverter952/1 -> VOUTP_Chkfin_flg/1  "VOUTP_Chkfin_flg"
  VTPM_SetIDLoc_flg/1 -> VTPM_SetIDLoc_flg_Inproc/1  "VTPM_SetIDLoc_flg"
  VTPM_SetIDLoc_flg_Inproc/1 -> UnitConverter953/1
  UnitConverter953/1 -> VOUTP_SetIDLoc_flg/1  "VOUTP_SetIDLoc_flg"
  VTPM_TPMSStorge_flg/1 -> VTPM_TPMSStorge_flg_Inproc/1  "VTPM_TPMSStorge_flg"
  VTPM_TPMSStorge_flg_Inproc/1 -> UnitConverter954/1
  UnitConverter954/1 -> VOUTP_TPMSStorge_flg/1  "VOUTP_TPMSStorge_flg"
  VTPM_ChkStorge_flg/1 -> VTPM_ChkStorge_flg_Inproc/1  "VTPM_ChkStorge_flg"
  VTPM_ChkStorge_flg_Inproc/1 -> UnitConverter955/1
  UnitConverter955/1 -> VOUTP_ChkStorge_flg/1  "VOUTP_ChkStorge_flg"
  VTPM_TPMSResButt_flg/1 -> VTPM_TPMSResButt_flg_Inproc/1  "VTPM_TPMSResButt_flg"
  VTPM_TPMSResButt_flg_Inproc/1 -> UnitConverter956/1
  UnitConverter956/1 -> VOUTP_TPMSResButt_flg/1  "VOUTP_TPMSResButt_flg"
  VTPM_LFPindi_enum/1 -> VTPM_LFPindi_enum_Inproc/1  "VTPM_LFPindi_enum"
  VTPM_LFPindi_enum_Inproc/1 -> UnitConverter957/1
  UnitConverter957/1 -> VOUTP_LFPindi_enum/1  "VOUTP_LFPindi_enum"
  VTPM_RFPind_enum/1 -> VTPM_RFPind_enum_Inproc/1  "VTPM_RFPind_enum"
  VTPM_RFPind_enum_Inproc/1 -> UnitConverter958/1
  UnitConverter958/1 -> VOUTP_RFPind_enum/1  "VOUTP_RFPind_enum"
  VTPM_LRPindi_enum/1 -> VTPM_LRPindi_enum_Inproc/1  "VTPM_LRPindi_enum"
  VTPM_LRPindi_enum_Inproc/1 -> UnitConverter959/1
  UnitConverter959/1 -> VOUTP_LRPindi_enum/1  "VOUTP_LRPindi_enum"
  VTPM_RRPindi_enum/1 -> VTPM_RRPindi_enum_Inproc/1  "VTPM_RRPindi_enum"
  VTPM_RRPindi_enum_Inproc/1 -> UnitConverter960/1
  UnitConverter960/1 -> VOUTP_RRPindi_enum/1  "VOUTP_RRPindi_enum"
  VTPM_WriteChkLFID_raw/1 -> VTPM_WriteChkLFID_raw_Inproc/1  "VTPM_WriteChkLFID_raw"
  VTPM_WriteChkLFID_raw_Inproc/1 -> UnitConverter961/1
  UnitConverter961/1 -> VOUTP_WriteChkLFID_raw/1  "VOUTP_WriteChkLFID_raw"
  VTPM_WriteChkRFID_raw/1 -> VTPM_WriteChkRFID_raw_Inproc/1  "VTPM_WriteChkRFID_raw"
  VTPM_WriteChkRFID_raw_Inproc/1 -> UnitConverter962/1
  UnitConverter962/1 -> VOUTP_WriteChkRFID_raw/1  "VOUTP_WriteChkRFID_raw"
  VTPM_WriteChkLRID_raw/1 -> VTPM_WriteChkLRID_raw_Inproc/1  "VTPM_WriteChkLRID_raw"
  VTPM_WriteChkLRID_raw_Inproc/1 -> UnitConverter963/1
  UnitConverter963/1 -> VOUTP_WriteChkLRID_raw/1  "VOUTP_WriteChkLRID_raw"
  VTPM_WriteChkRRID_raw/1 -> VTPM_WriteChkRRID_raw_Inproc/1  "VTPM_WriteChkRRID_raw"
  VTPM_WriteChkRRID_raw_Inproc/1 -> UnitConverter964/1
  UnitConverter964/1 -> VOUTP_WriteChkRRID_raw/1  "VOUTP_WriteChkRRID_raw"
  VTPM_WriteChkfinLFID_raw/1 -> VTPM_WriteChkfinLFID_raw_Inproc/1  "VTPM_WriteChkfinLFID_raw"
  VTPM_WriteChkfinLFID_raw_Inproc/1 -> UnitConverter965/1
  UnitConverter965/1 -> VOUTP_WriteChkfinLFID_raw/1  "VOUTP_WriteChkfinLFID_raw"
  VTPM_WriteChkfinRFID_raw/1 -> VTPM_WriteChkfinRFID_raw_Inproc/1  "VTPM_WriteChkfinRFID_raw"
  VTPM_WriteChkfinRFID_raw_Inproc/1 -> UnitConverter966/1
  UnitConverter966/1 -> VOUTP_WriteChkfinRFID_raw/1  "VOUTP_WriteChkfinRFID_raw"
  VTPM_WriteChkfinLRID_raw/1 -> VTPM_WriteChkfinLRID_raw_Inproc/1  "VTPM_WriteChkfinLRID_raw"
  VTPM_WriteChkfinLRID_raw_Inproc/1 -> UnitConverter967/1
  UnitConverter967/1 -> VOUTP_WriteChkfinLRID_raw/1  "VOUTP_WriteChkfinLRID_raw"
  VTPM_WriteChkfinRRID_raw/1 -> VTPM_WriteChkfinRRID_raw_Inproc/1  "VTPM_WriteChkfinRRID_raw"
  VTPM_WriteChkfinRRID_raw_Inproc/1 -> UnitConverter968/1
  UnitConverter968/1 -> VOUTP_WriteChkfinRRID_raw/1  "VOUTP_WriteChkfinRRID_raw"
  VTPM_Flashchkdatavalid_enum/1 -> VTPM_Flashchkdatavalid_enum_Inproc/1  "VTPM_Flashchkdatavalid_enum"
  VTPM_Flashchkdatavalid_enum_Inproc/1 -> UnitConverter969/1
  UnitConverter969/1 -> VOUTP_Flashchkdatavalid_enum/1  "VOUTP_Flashchkdatavalid_enum"
  VTPM_Flashdatavalid_enum/1 -> VTPM_Flashdatavalid_enum_Inproc/1  "VTPM_Flashdatavalid_enum"
  VTPM_Flashdatavalid_enum_Inproc/1 -> UnitConverter970/1
  UnitConverter970/1 -> VOUTP_Flashdatavalid_enum/1  "VOUTP_Flashdatavalid_enum"
  VTPM_unlearnSfali_flg/1 -> VTPM_unlearnSfali_flg_Inproc/1  "VTPM_unlearnSfali_flg"
  VTPM_unlearnSfali_flg_Inproc/1 -> UnitConverter971/1
  UnitConverter971/1 -> VOUTP_unlearnSfali_flg/1  "VOUTP_unlearnSfali_flg"
  VTPM_unlearnSfailvalid_enum/1 -> VTPM_unlearnSfailvalid_enum_Inproc/1  "VTPM_unlearnSfailvalid_enum"
  VTPM_unlearnSfailvalid_enum_Inproc/1 -> UnitConverter972/1
  UnitConverter972/1 -> VOUTP_unlearnSfailvalid_enum/1  "VOUTP_unlearnSfailvalid_enum"
  VTPM_Prepresstempvalid_enum/1 -> VTPM_Prepresstempvalid_enum_Inproc/1  "VTPM_Prepresstempvalid_enum"
  VTPM_Prepresstempvalid_enum_Inproc/1 -> UnitConverter973/1
  UnitConverter973/1 -> VOUTP_Prepresstempvalid_enum/1  "VOUTP_Prepresstempvalid_enum"
  VTPM_FlashS1ID_raw/1 -> VTPM_FlashS1ID_raw_Inproc/1  "VTPM_FlashS1ID_raw"
  VTPM_FlashS1ID_raw_Inproc/1 -> UnitConverter974/1
  UnitConverter974/1 -> VOUTP_FlashS1ID_raw/1  "VOUTP_FlashS1ID_raw"
  VTPM_FlashS2ID_raw/1 -> VTPM_FlashS2ID_raw_Inproc/1  "VTPM_FlashS2ID_raw"
  VTPM_FlashS2ID_raw_Inproc/1 -> UnitConverter975/1
  UnitConverter975/1 -> VOUTP_FlashS2ID_raw/1  "VOUTP_FlashS2ID_raw"
  VTPM_FlashS3ID_raw/1 -> VTPM_FlashS3ID_raw_Inproc/1  "VTPM_FlashS3ID_raw"
  VTPM_FlashS3ID_raw_Inproc/1 -> UnitConverter976/1
  UnitConverter976/1 -> VOUTP_FlashS3ID_raw/1  "VOUTP_FlashS3ID_raw"
  VTPM_FlashS4ID_raw/1 -> VTPM_FlashS4ID_raw_Inproc/1  "VTPM_FlashS4ID_raw"
  VTPM_FlashS4ID_raw_Inproc/1 -> UnitConverter977/1
  UnitConverter977/1 -> VOUTP_FlashS4ID_raw/1  "VOUTP_FlashS4ID_raw"
  VTPM_FlashIDvalid_enum/1 -> VTPM_FlashIDvalid_enum_Inproc/1  "VTPM_FlashIDvalid_enum"
  VTPM_FlashIDvalid_enum_Inproc/1 -> UnitConverter978/1
  UnitConverter978/1 -> VOUTP_FlashIDvalid_enum/1  "VOUTP_FlashIDvalid_enum"
  VTPM_WritingCnt_enum/1 -> VTPM_WritingCnt_enum_Inproc/1  "VTPM_WritingCnt_enum"
  VTPM_WritingCnt_enum_Inproc/1 -> UnitConverter979/1
  UnitConverter979/1 -> VOUTP_WritingCnt_enum/1  "VOUTP_WritingCnt_enum"
  VTPM_TPMSTLCmd_flg/1 -> VTPM_TPMSTLCmd_flg_Inproc/1  "VTPM_TPMSTLCmd_flg"
  VTPM_TPMSTLCmd_flg_Inproc/1 -> UnitConverter980/1
  UnitConverter980/1 -> VOUTP_TPMSTLCmd_flg/1  "VOUTP_TPMSTLCmd_flg"
  VTPM_LProgress_enum/1 -> VTPM_LProgress_enum_Inproc/1  "VTPM_LProgress_enum"
  VTPM_LProgress_enum_Inproc/1 -> UnitConverter981/1
  UnitConverter981/1 -> VOUTP_LProgress_enum/1  "VOUTP_LProgress_enum"
  VTPM_TPMSSensorIDRegStart_flg/1 -> VTPM_TPMSSensorIDRegStart_flg_Inproc/1  "VTPM_TPMSSensorIDRegStart_flg"
  VTPM_TPMSSensorIDRegStart_flg_Inproc/1 -> UnitConverter982/1
  UnitConverter982/1 -> VOUTP_TPMSSensorIDRegStart_flg/1  "VOUTP_TPMSSensorIDRegStart_flg"
  VTPM_ModelVersion_raw/1 -> VTPM_ModelVersion_raw_Inproc/1  "VTPM_ModelVersion_raw"
  VTPM_ModelVersion_raw_Inproc/1 -> UnitConverter983/1
  UnitConverter983/1 -> VOUTP_ModelVersion_raw/1  "VOUTP_ModelVersion_raw"
  VTPM_ModelVersionChksum_raw/1 -> VTPM_ModelVersionChksum_raw_Inproc/1  "VTPM_ModelVersionChksum_raw"
  VTPM_ModelVersionChksum_raw_Inproc/1 -> UnitConverter984/1
  UnitConverter984/1 -> VOUTP_ModelVersionChksum_raw/1  "VOUTP_ModelVersionChksum_raw"
  VTQD_ParkRequest_flg/1 -> VTQD_ParkRequest_flg_Inproc/1  "VTQD_ParkRequest_flg"
  VTQD_ParkRequest_flg_Inproc/1 -> UnitConverter985/1
  UnitConverter985/1 -> VOUTP_ParkRequest_flg/1  "VOUTP_ParkRequest_flg"
  VTQD_TqSourceFr_enum/1 -> VTQD_TqSourceFr_enum_Inproc/1  "VTQD_TqSourceFr_enum"
  VTQD_TqSourceFr_enum_Inproc/1 -> UnitConverter986/1
  UnitConverter986/1 -> VOUTP_TqSourceFr_enum/1  "VOUTP_TqSourceFr_enum"
  VTQD_TqSourceRr_enum/1 -> VTQD_TqSourceRr_enum_Inproc/1  "VTQD_TqSourceRr_enum"
  VTQD_TqSourceRr_enum_Inproc/1 -> UnitConverter987/1
  UnitConverter987/1 -> VOUTP_TqSourceRr_enum/1  "VOUTP_TqSourceRr_enum"
  VTQD_FrEDUAvailBrkRgnTq_Nm/1 -> VTQD_FrEDUAvailBrkRgnTq_Nm_Inproc/1  "VTQD_FrEDUAvailBrkRgnTq_Nm"
  VTQD_FrEDUAvailBrkRgnTq_Nm_Inproc/1 -> UnitConverter988/1
  UnitConverter988/1 -> VOUTP_FrEDUAvailBrkRgnTq_Nm/1  "VOUTP_FrEDUAvailBrkRgnTq_Nm"
  VTQD_RrEDUAvailBrkRgnTq_Nm/1 -> VTQD_RrEDUAvailBrkRgnTq_Nm_Inproc/1  "VTQD_RrEDUAvailBrkRgnTq_Nm"
  VTQD_RrEDUAvailBrkRgnTq_Nm_Inproc/1 -> UnitConverter989/1
  UnitConverter989/1 -> VOUTP_RrEDUAvailBrkRgnTq_Nm/1  "VOUTP_RrEDUAvailBrkRgnTq_Nm"
  VTQD_EVDriveMode_enum/1 -> VTQD_EVDriveMode_enum_Inproc/1  "VTQD_EVDriveMode_enum"
  VTQD_EVDriveMode_enum_Inproc/1 -> UnitConverter990/1
  UnitConverter990/1 -> VOUTP_EVDriveMode_enum/1  "VOUTP_EVDriveMode_enum"
  VTQD_ShiftGearPosn_enum/1 -> VTQD_ShiftGearPosn_enum_Inproc/1  "VTQD_ShiftGearPosn_enum"
  VTQD_ShiftGearPosn_enum_Inproc/1 -> UnitConverter991/1
  UnitConverter991/1 -> VOUTP_ShiftGearPosn_enum/1  "VOUTP_ShiftGearPosn_enum"
  VTQD_PButtonSta_enum/1 -> VTQD_PButtonSta_enum_Inproc/1  "VTQD_PButtonSta_enum"
  VTQD_PButtonSta_enum_Inproc/1 -> UnitConverter992/1
  UnitConverter992/1 -> VOUTP_PButtonSta_enum/1  "VOUTP_PButtonSta_enum"
  VTQD_FrActvDmpDisabReq_flg/1 -> VTQD_FrActvDmpDisabReq_flg_Inproc/1  "VTQD_FrActvDmpDisabReq_flg"
  VTQD_FrActvDmpDisabReq_flg_Inproc/1 -> UnitConverter993/1
  UnitConverter993/1 -> VOUTP_FrActvDmpDisabReq_flg/1  "VOUTP_FrActvDmpDisabReq_flg"
  VTQD_RrActvDmpDisabReq_flg/1 -> VTQD_RrActvDmpDisabReq_flg_Inproc/1  "VTQD_RrActvDmpDisabReq_flg"
  VTQD_RrActvDmpDisabReq_flg_Inproc/1 -> UnitConverter994/1
  UnitConverter994/1 -> VOUTP_RrActvDmpDisabReq_flg/1  "VOUTP_RrActvDmpDisabReq_flg"
  VTQD_FrRgnDecrSta_flg/1 -> VTQD_FrRgnDecrSta_flg_Inproc/1  "VTQD_FrRgnDecrSta_flg"
  VTQD_FrRgnDecrSta_flg_Inproc/1 -> UnitConverter995/1
  UnitConverter995/1 -> VOUTP_FrRgnDecrSta_flg/1  "VOUTP_FrRgnDecrSta_flg"
  VTQD_RrRgnDecrSta_flg/1 -> VTQD_RrRgnDecrSta_flg_Inproc/1  "VTQD_RrRgnDecrSta_flg"
  VTQD_RrRgnDecrSta_flg_Inproc/1 -> UnitConverter996/1
  UnitConverter996/1 -> VOUTP_RrRgnDecrSta_flg/1  "VOUTP_RrRgnDecrSta_flg"
  VTQD_DriverWhlTqDemFr_Nm/1 -> VTQD_DriverWhlTqDemFr_Nm_Inproc/1  "VTQD_DriverWhlTqDemFr_Nm"
  VTQD_DriverWhlTqDemFr_Nm_Inproc/1 -> UnitConverter997/1
  UnitConverter997/1 -> VOUTP_DriverWhlTqDemFr_Nm/1  "VOUTP_DriverWhlTqDemFr_Nm"
  VTQD_DriverWhlTqDemRr_Nm/1 -> VTQD_DriverWhlTqDemRr_Nm_Inproc/1  "VTQD_DriverWhlTqDemRr_Nm"
  VTQD_DriverWhlTqDemRr_Nm_Inproc/1 -> UnitConverter998/1
  UnitConverter998/1 -> VOUTP_DriverWhlTqDemRr_Nm/1  "VOUTP_DriverWhlTqDemRr_Nm"
  VTQD_FrEDUActTq_Nm/1 -> VTQD_FrEDUActTq_Nm_Inproc/1  "VTQD_FrEDUActTq_Nm"
  VTQD_FrEDUActTq_Nm_Inproc/1 -> UnitConverter999/1
  UnitConverter999/1 -> VOUTP_FrEDUActTq_Nm/1  "VOUTP_FrEDUActTq_Nm"
  VTQD_RrEDUActTq_Nm/1 -> VTQD_RrEDUActTq_Nm_Inproc/1  "VTQD_RrEDUActTq_Nm"
  VTQD_RrEDUActTq_Nm_Inproc/1 -> UnitConverter1000/1
  UnitConverter1000/1 -> VOUTP_RrEDUActTq_Nm/1  "VOUTP_RrEDUActTq_Nm"
  VTQD_FrEDURolRgnTq_Nm/1 -> VTQD_FrEDURolRgnTq_Nm_Inproc/1  "VTQD_FrEDURolRgnTq_Nm"
  VTQD_FrEDURolRgnTq_Nm_Inproc/1 -> UnitConverter1001/1
  UnitConverter1001/1 -> VOUTP_FrEDURolRgnTq_Nm/1  "VOUTP_FrEDURolRgnTq_Nm"
  VTQD_RrEDURolRgnTq_Nm/1 -> VTQD_RrEDURolRgnTq_Nm_Inproc/1  "VTQD_RrEDURolRgnTq_Nm"
  VTQD_RrEDURolRgnTq_Nm_Inproc/1 -> UnitConverter1002/1
  UnitConverter1002/1 -> VOUTP_RrEDURolRgnTq_Nm/1  "VOUTP_RrEDURolRgnTq_Nm"
  VTQD_FrEDUSpd_rpm/1 -> VTQD_FrEDUSpd_rpm_Inproc/1  "VTQD_FrEDUSpd_rpm"
  VTQD_FrEDUSpd_rpm_Inproc/1 -> UnitConverter1003/1
  UnitConverter1003/1 -> VOUTP_FrEDUSpd_rpm/1  "VOUTP_FrEDUSpd_rpm"
  VTQD_RrEDUSpd_rpm/1 -> VTQD_RrEDUSpd_rpm_Inproc/1  "VTQD_RrEDUSpd_rpm"
  VTQD_RrEDUSpd_rpm_Inproc/1 -> UnitConverter1004/1
  UnitConverter1004/1 -> VOUTP_RrEDUSpd_rpm/1  "VOUTP_RrEDUSpd_rpm"
  VTQD_FrEDUSpdValid_flg/1 -> VTQD_FrEDUSpdValid_flg_Inproc/1  "VTQD_FrEDUSpdValid_flg"
  VTQD_FrEDUSpdValid_flg_Inproc/1 -> UnitConverter1005/1
  UnitConverter1005/1 -> VOUTP_FrEDUSpdValid_flg/1  "VOUTP_FrEDUSpdValid_flg"
  VTQD_FrEDUAvailBrkRgnTqV_flg/1 -> VTQD_FrEDUAvailBrkRgnTqV_flg_Inproc/1  "VTQD_FrEDUAvailBrkRgnTqV_flg"
  VTQD_FrEDUAvailBrkRgnTqV_flg_Inproc/1 -> UnitConverter1006/1
  UnitConverter1006/1 -> VOUTP_FrEDUAvailBrkRgnTqV_flg/1  "VOUTP_FrEDUAvailBrkRgnTqV_flg"
  VTQD_RrEDUSpdValid_flg/1 -> VTQD_RrEDUSpdValid_flg_Inproc/1  "VTQD_RrEDUSpdValid_flg"
  VTQD_RrEDUSpdValid_flg_Inproc/1 -> UnitConverter1007/1
  UnitConverter1007/1 -> VOUTP_RrEDUSpdValid_flg/1  "VOUTP_RrEDUSpdValid_flg"
  VTQD_RrEDUAvailBrkRgnTqV_flg/1 -> VTQD_RrEDUAvailBrkRgnTqV_flg_Inproc/1  "VTQD_RrEDUAvailBrkRgnTqV_flg"
  VTQD_RrEDUAvailBrkRgnTqV_flg_Inproc/1 -> UnitConverter1008/1
  UnitConverter1008/1 -> VOUTP_RrEDUAvailBrkRgnTqV_flg/1  "VOUTP_RrEDUAvailBrkRgnTqV_flg"
  VTQD_RgnAbnorSta_flg/1 -> VTQD_RgnAbnorSta_flg_Inproc/1  "VTQD_RgnAbnorSta_flg"
  VTQD_RgnAbnorSta_flg_Inproc/1 -> UnitConverter1009/1
  UnitConverter1009/1 -> VOUTP_RgnAbnorSta_flg/1  "VOUTP_RgnAbnorSta_flg"
  VTQD_PTCSPermSta_flg/1 -> VTQD_PTCSPermSta_flg_Inproc/1  "VTQD_PTCSPermSta_flg"
  VTQD_PTCSPermSta_flg_Inproc/1 -> UnitConverter1010/1
  UnitConverter1010/1 -> VOUTP_PTCSPermSta_flg/1  "VOUTP_PTCSPermSta_flg"
  VTQD_FrRgnPermSta_flg/1 -> VTQD_FrRgnPermSta_flg_Inproc/1  "VTQD_FrRgnPermSta_flg"
  VTQD_FrRgnPermSta_flg_Inproc/1 -> UnitConverter1011/1
  UnitConverter1011/1 -> VOUTP_FrRgnPermSta_flg/1  "VOUTP_FrRgnPermSta_flg"
  VTQD_RrRgnPermSta_flg/1 -> VTQD_RrRgnPermSta_flg_Inproc/1  "VTQD_RrRgnPermSta_flg"
  VTQD_RrRgnPermSta_flg_Inproc/1 -> UnitConverter1012/1
  UnitConverter1012/1 -> VOUTP_RrRgnPermSta_flg/1  "VOUTP_RrRgnPermSta_flg"
  VTQD_FrIdcMin_A/1 -> VTQD_FrIdcMin_A_Inproc/1  "VTQD_FrIdcMin_A"
  VTQD_FrIdcMin_A_Inproc/1 -> UnitConverter1013/1
  UnitConverter1013/1 -> VOUTP_FrIdcMin_A/1  "VOUTP_FrIdcMin_A"
  VTQD_FrIdcMax_A/1 -> VTQD_FrIdcMax_A_Inproc/1  "VTQD_FrIdcMax_A"
  VTQD_FrIdcMax_A_Inproc/1 -> UnitConverter1014/1
  UnitConverter1014/1 -> VOUTP_FrIdcMax_A/1  "VOUTP_FrIdcMax_A"
  VTQD_FrUdcMin_V/1 -> VTQD_FrUdcMin_V_Inproc/1  "VTQD_FrUdcMin_V"
  VTQD_FrUdcMin_V_Inproc/1 -> UnitConverter1015/1
  UnitConverter1015/1 -> VOUTP_FrUdcMin_V/1  "VOUTP_FrUdcMin_V"
  VTQD_FrUdcMax_V/1 -> VTQD_FrUdcMax_V_Inproc/1  "VTQD_FrUdcMax_V"
  VTQD_FrUdcMax_V_Inproc/1 -> UnitConverter1016/1
  UnitConverter1016/1 -> VOUTP_FrUdcMax_V/1  "VOUTP_FrUdcMax_V"
  VTQD_RrIdcMin_A/1 -> VTQD_RrIdcMin_A_Inproc/1  "VTQD_RrIdcMin_A"
  VTQD_RrIdcMin_A_Inproc/1 -> UnitConverter1017/1
  UnitConverter1017/1 -> VOUTP_RrIdcMin_A/1  "VOUTP_RrIdcMin_A"
  VTQD_RrIdcMax_A/1 -> VTQD_RrIdcMax_A_Inproc/1  "VTQD_RrIdcMax_A"
  VTQD_RrIdcMax_A_Inproc/1 -> UnitConverter1018/1
  UnitConverter1018/1 -> VOUTP_RrIdcMax_A/1  "VOUTP_RrIdcMax_A"
  VTQD_RrUdcMin_V/1 -> VTQD_RrUdcMin_V_Inproc/1  "VTQD_RrUdcMin_V"
  VTQD_RrUdcMin_V_Inproc/1 -> UnitConverter1019/1
  UnitConverter1019/1 -> VOUTP_RrUdcMin_V/1  "VOUTP_RrUdcMin_V"
  VTQD_RrUdcMax_V/1 -> VTQD_RrUdcMax_V_Inproc/1  "VTQD_RrUdcMax_V"
  VTQD_RrUdcMax_V_Inproc/1 -> UnitConverter1020/1
  UnitConverter1020/1 -> VOUTP_RrUdcMax_V/1  "VOUTP_RrUdcMax_V"
  VTQD_ReBrakeLPReq_flg/1 -> VTQD_ReBrakeLPReq_flg_Inproc/1  "VTQD_ReBrakeLPReq_flg"
  VTQD_ReBrakeLPReq_flg_Inproc/1 -> UnitConverter1021/1
  UnitConverter1021/1 -> VOUTP_ReBrakeLPReq_flg/1  "VOUTP_ReBrakeLPReq_flg"
  VTQD_BOSEnable_flg/1 -> VTQD_BOSEnable_flg_Inproc/1  "VTQD_BOSEnable_flg"
  VTQD_BOSEnable_flg_Inproc/1 -> UnitConverter1022/1
  UnitConverter1022/1 -> VOUTP_BOSEnable_flg/1  "VOUTP_BOSEnable_flg"
  VTQD_CreepON_flg/1 -> VTQD_CreepON_flg_Inproc/1  "VTQD_CreepON_flg"
  VTQD_CreepON_flg_Inproc/1 -> UnitConverter1023/1
  UnitConverter1023/1 -> VOUTP_CreepON_flg/1  "VOUTP_CreepON_flg"
  VTQD_RDCActive_enum/1 -> VTQD_RDCActive_enum_Inproc/1  "VTQD_RDCActive_enum"
  VTQD_RDCActive_enum_Inproc/1 -> UnitConverter1024/1
  UnitConverter1024/1 -> VOUTP_RDCActive_enum/1  "VOUTP_RDCActive_enum"
  VTQD_EquivAccPedalSWSta_flg/1 -> VTQD_EquivAccPedalSWSta_flg_Inproc/1  "VTQD_EquivAccPedalSWSta_flg"
  VTQD_EquivAccPedalSWSta_flg_Inproc/1 -> UnitConverter1025/1
  UnitConverter1025/1 -> VOUTP_EquivAccPedalSWSta_flg/1  "VOUTP_EquivAccPedalSWSta_flg"
  VTQD_DriveProtEn_flg/1 -> VTQD_DriveProtEn_flg_Inproc/1  "VTQD_DriveProtEn_flg"
  VTQD_DriveProtEn_flg_Inproc/1 -> UnitConverter1026/1
  UnitConverter1026/1 -> VOUTP_DriveProtEn_flg/1  "VOUTP_DriveProtEn_flg"
  VTQD_ActParkRequest_flg/1 -> VTQD_ActParkRequest_flg_Inproc/1  "VTQD_ActParkRequest_flg"
  VTQD_ActParkRequest_flg_Inproc/1 -> UnitConverter1027/1
  UnitConverter1027/1 -> VOUTP_ActParkRequest_flg/1  "VOUTP_ActParkRequest_flg"
  VTQD_RegenTqLimitEn_flg/1 -> VTQD_RegenTqLimitEn_flg_Inproc/1  "VTQD_RegenTqLimitEn_flg"
  VTQD_RegenTqLimitEn_flg_Inproc/1 -> UnitConverter1028/1
  UnitConverter1028/1 -> VOUTP_RegenTqLimitEn_flg/1  "VOUTP_RegenTqLimitEn_flg"
  VTQD_IVIPwrLockSta_enum/1 -> VTQD_IVIPwrLockSta_enum_Inproc/1  "VTQD_IVIPwrLockSta_enum"
  VTQD_IVIPwrLockSta_enum_Inproc/1 -> UnitConverter1029/1
  UnitConverter1029/1 -> VOUTP_IVIPwrLockSta_enum/1  "VOUTP_IVIPwrLockSta_enum"
  VTQD_OPDHoldLamp_flg/1 -> VTQD_OPDHoldLamp_flg_Inproc/1  "VTQD_OPDHoldLamp_flg"
  VTQD_OPDHoldLamp_flg_Inproc/1 -> UnitConverter1030/1
  UnitConverter1030/1 -> VOUTP_OPDHoldLamp_flg/1  "VOUTP_OPDHoldLamp_flg"
  VTQD_SaveRegenMode_enum/1 -> VTQD_SaveRegenMode_enum_Inproc/1  "VTQD_SaveRegenMode_enum"
  VTQD_SaveRegenMode_enum_Inproc/1 -> UnitConverter1031/1
  UnitConverter1031/1 -> VOUTP_SaveRegenMode_enum/1  "VOUTP_SaveRegenMode_enum"
  VTQD_FDCVCURegenMode_enum/1 -> VTQD_FDCVCURegenMode_enum_Inproc/1  "VTQD_FDCVCURegenMode_enum"
  VTQD_FDCVCURegenMode_enum_Inproc/1 -> UnitConverter1032/1
  UnitConverter1032/1 -> VOUTP_FDCVCURegenMode_enum/1  "VOUTP_FDCVCURegenMode_enum"
  VTQD_SpdCtrlMode_enum/1 -> VTQD_SpdCtrlMode_enum_Inproc/1  "VTQD_SpdCtrlMode_enum"
  VTQD_SpdCtrlMode_enum_Inproc/1 -> UnitConverter1033/1
  UnitConverter1033/1 -> VOUTP_SpdCtrlMode_enum/1  "VOUTP_SpdCtrlMode_enum"
  VTQD_SpdCtrlSta_flg/1 -> VTQD_SpdCtrlSta_flg_Inproc/1  "VTQD_SpdCtrlSta_flg"
  VTQD_SpdCtrlSta_flg_Inproc/1 -> UnitConverter1034/1
  UnitConverter1034/1 -> VOUTP_SpdCtrlSta_flg/1  "VOUTP_SpdCtrlSta_flg"
  VTQD_SetSpd_kph/1 -> VTQD_SetSpd_kph_Inproc/1  "VTQD_SetSpd_kph"
  VTQD_SetSpd_kph_Inproc/1 -> UnitConverter1035/1
  UnitConverter1035/1 -> VOUTP_SetSpd_kph/1  "VOUTP_SetSpd_kph"
  VTQD_VehActSpd_kph/1 -> VTQD_VehActSpd_kph_Inproc/1  "VTQD_VehActSpd_kph"
  VTQD_VehActSpd_kph_Inproc/1 -> UnitConverter1036/1
  UnitConverter1036/1 -> VOUTP_VehActSpd_kph/1  "VOUTP_VehActSpd_kph"
  VTQD_RegenLimIndSta_flg/1 -> VTQD_RegenLimIndSta_flg_Inproc/1  "VTQD_RegenLimIndSta_flg"
  VTQD_RegenLimIndSta_flg_Inproc/1 -> UnitConverter1037/1
  UnitConverter1037/1 -> VOUTP_RegenLimIndSta_flg/1  "VOUTP_RegenLimIndSta_flg"
  VTQD_SetSpdLimWarn_flg/1 -> VTQD_SetSpdLimWarn_flg_Inproc/1  "VTQD_SetSpdLimWarn_flg"
  VTQD_SetSpdLimWarn_flg_Inproc/1 -> UnitConverter1038/1
  UnitConverter1038/1 -> VOUTP_SetSpdLimWarn_flg/1  "VOUTP_SetSpdLimWarn_flg"
  VTQD_MaxWhlSlideRate_pct/1 -> VTQD_MaxWhlSlideRate_pct_Inproc/1  "VTQD_MaxWhlSlideRate_pct"
  VTQD_MaxWhlSlideRate_pct_Inproc/1 -> UnitConverter1039/1
  UnitConverter1039/1 -> VOUTP_MaxWhlSlideRate_pct/1  "VOUTP_MaxWhlSlideRate_pct"
  VTQD_TrailerDisOPDSta_flg/1 -> VTQD_TrailerDisOPDSta_flg_Inproc/1  "VTQD_TrailerDisOPDSta_flg"
  VTQD_TrailerDisOPDSta_flg_Inproc/1 -> UnitConverter1040/1
  UnitConverter1040/1 -> VOUTP_TrailerDisOPDSta_flg/1  "VOUTP_TrailerDisOPDSta_flg"
  VTQD_ForceP_flg/1 -> VTQD_ForceP_flg_Inproc/1  "VTQD_ForceP_flg"
  VTQD_ForceP_flg_Inproc/1 -> UnitConverter1041/1
  UnitConverter1041/1 -> VOUTP_ForceP_flg/1  "VOUTP_ForceP_flg"
  VTQD_SlideRegenLimTq_Nm/1 -> VTQD_SlideRegenLimTq_Nm_Inproc/1  "VTQD_SlideRegenLimTq_Nm"
  VTQD_SlideRegenLimTq_Nm_Inproc/1 -> UnitConverter1042/1
  UnitConverter1042/1 -> VOUTP_SlideRegenLimTq_Nm/1  "VOUTP_SlideRegenLimTq_Nm"
  VTQD_SimSoundCmd_pct/1 -> VTQD_SimSoundCmd_pct_Inproc/1  "VTQD_SimSoundCmd_pct"
  VTQD_SimSoundCmd_pct_Inproc/1 -> UnitConverter1043/1
  UnitConverter1043/1 -> VOUTP_SimSoundCmd_pct/1  "VOUTP_SimSoundCmd_pct"
  VTQD_SimSouWaveReq_pct/1 -> VTQD_SimSouWaveReq_pct_Inproc/1  "VTQD_SimSouWaveReq_pct"
  VTQD_SimSouWaveReq_pct_Inproc/1 -> UnitConverter1044/1
  UnitConverter1044/1 -> VOUTP_SimSouWaveReq_pct/1  "VOUTP_SimSouWaveReq_pct"
  VTQR_FrTMTqReq_Nm/1 -> VTQR_FrTMTqReq_Nm_Inproc/1  "VTQR_FrTMTqReq_Nm"
  VTQR_FrTMTqReq_Nm_Inproc/1 -> UnitConverter1045/1
  UnitConverter1045/1 -> VOUTP_FrTMTqReq_Nm/1  "VOUTP_FrTMTqReq_Nm"
  VTQR_RrTMTqReq_Nm/1 -> VTQR_RrTMTqReq_Nm_Inproc/1  "VTQR_RrTMTqReq_Nm"
  VTQR_RrTMTqReq_Nm_Inproc/1 -> UnitConverter1046/1
  UnitConverter1046/1 -> VOUTP_RrTMTqReq_Nm/1  "VOUTP_RrTMTqReq_Nm"
  VTQR_FrFirstOrderInpTs_c/1 -> VTQR_FrFirstOrderInpTs_c_Inproc/1  "VTQR_FrFirstOrderInpTs_c"
  VTQR_FrFirstOrderInpTs_c_Inproc/1 -> UnitConverter1047/1
  UnitConverter1047/1 -> VOUTP_FrFirstOrderInpTs_c/1  "VOUTP_FrFirstOrderInpTs_c"
  VTQR_RrFirstOrderInpTs_c/1 -> VTQR_RrFirstOrderInpTs_c_Inproc/1  "VTQR_RrFirstOrderInpTs_c"
  VTQR_RrFirstOrderInpTs_c_Inproc/1 -> UnitConverter1048/1
  UnitConverter1048/1 -> VOUTP_RrFirstOrderInpTs_c/1  "VOUTP_RrFirstOrderInpTs_c"
  VTQR_FrRateLimitInc_Nm/1 -> VTQR_FrRateLimitInc_Nm_Inproc/1  "VTQR_FrRateLimitInc_Nm"
  VTQR_FrRateLimitInc_Nm_Inproc/1 -> UnitConverter1049/1
  UnitConverter1049/1 -> VOUTP_FrRateLimitInc_Nm/1  "VOUTP_FrRateLimitInc_Nm"
  VTQR_FrRateLimitDec_Nm/1 -> VTQR_FrRateLimitDec_Nm_Inproc/1  "VTQR_FrRateLimitDec_Nm"
  VTQR_FrRateLimitDec_Nm_Inproc/1 -> UnitConverter1050/1
  UnitConverter1050/1 -> VOUTP_FrRateLimitDec_Nm/1  "VOUTP_FrRateLimitDec_Nm"
  VTQR_RrRateLimitInc_Nm/1 -> VTQR_RrRateLimitInc_Nm_Inproc/1  "VTQR_RrRateLimitInc_Nm"
  VTQR_RrRateLimitInc_Nm_Inproc/1 -> UnitConverter1051/1
  UnitConverter1051/1 -> VOUTP_RrRateLimitInc_Nm/1  "VOUTP_RrRateLimitInc_Nm"
  VTQR_RrRateLimitDec_Nm/1 -> VTQR_RrRateLimitDec_Nm_Inproc/1  "VTQR_RrRateLimitDec_Nm"
  VTQR_RrRateLimitDec_Nm_Inproc/1 -> UnitConverter1052/1
  UnitConverter1052/1 -> VOUTP_RrRateLimitDec_Nm/1  "VOUTP_RrRateLimitDec_Nm"
  VV2L_ReqOBCV2LEna_enum/1 -> VV2L_ReqOBCV2LEna_enum_Inproc/1  "VV2L_ReqOBCV2LEna_enum"
  VV2L_ReqOBCV2LEna_enum_Inproc/1 -> UnitConverter1053/1
  UnitConverter1053/1 -> VOUTP_ReqOBCV2LEna_enum/1  "VOUTP_ReqOBCV2LEna_enum"
  VV2L_ReqV2LIVIPopup_enum/1 -> VV2L_ReqV2LIVIPopup_enum_Inproc/1  "VV2L_ReqV2LIVIPopup_enum"
  VV2L_ReqV2LIVIPopup_enum_Inproc/1 -> UnitConverter1054/1
  UnitConverter1054/1 -> VOUTP_ReqV2LIVIPopup_enum/1  "VOUTP_ReqV2LIVIPopup_enum"
  VV2L_ReqV2LIVIDisChrg_enum/1 -> VV2L_ReqV2LIVIDisChrg_enum_Inproc/1  "VV2L_ReqV2LIVIDisChrg_enum"
  VV2L_ReqV2LIVIDisChrg_enum_Inproc/1 -> UnitConverter1055/1
  UnitConverter1055/1 -> VOUTP_ReqV2LIVIDisChrg_enum/1  "VOUTP_ReqV2LIVIDisChrg_enum"
  VV2L_ReqOBCExtrV2LEna_enum/1 -> VV2L_ReqOBCExtrV2LEna_enum_Inproc/1  "VV2L_ReqOBCExtrV2LEna_enum"
  VV2L_ReqOBCExtrV2LEna_enum_Inproc/1 -> UnitConverter1056/1
  UnitConverter1056/1 -> VOUTP_ReqOBCExtrV2LEna_enum/1  "VOUTP_ReqOBCExtrV2LEna_enum"
  VV2L_ReqOBCIntrV2LEna_enum/1 -> VV2L_ReqOBCIntrV2LEna_enum_Inproc/1  "VV2L_ReqOBCIntrV2LEna_enum"
  VV2L_ReqOBCIntrV2LEna_enum_Inproc/1 -> UnitConverter1057/1
  UnitConverter1057/1 -> VOUTP_ReqOBCIntrV2LEna_enum/1  "VOUTP_ReqOBCIntrV2LEna_enum"
  VV2L_HVPO120VGrpALDSt_enum/1 -> VV2L_HVPO120VGrpALDSt_enum_Inproc/1  "VV2L_HVPO120VGrpALDSt_enum"
  VV2L_HVPO120VGrpALDSt_enum_Inproc/1 -> UnitConverter1058/1
  UnitConverter1058/1 -> VOUTP_HVPO120VGrpALDSt_enum/1  "VOUTP_HVPO120VGrpALDSt_enum"
  VV2L_HVPO120VGrpBLDSt_enum/1 -> VV2L_HVPO120VGrpBLDSt_enum_Inproc/1  "VV2L_HVPO120VGrpBLDSt_enum"
  VV2L_HVPO120VGrpBLDSt_enum_Inproc/1 -> UnitConverter1059/1
  UnitConverter1059/1 -> VOUTP_HVPO120VGrpBLDSt_enum/1  "VOUTP_HVPO120VGrpBLDSt_enum"
  VVMC_FeatSetSpdFinal_raw32/1 -> VVMC_FeatSetSpdFinal_raw32_Inproc/1  "VVMC_FeatSetSpdFinal_raw32"
  VVMC_FeatSetSpdFinal_raw32_Inproc/1 -> UnitConverter1060/1
  UnitConverter1060/1 -> VOUTP_FeatSetSpdFinal_raw32/1  "VOUTP_FeatSetSpdFinal_raw32"
  VVMC_VehicleSpeed_mph/1 -> VVMC_VehicleSpeed_mph_Inproc/1  "VVMC_VehicleSpeed_mph"
  VVMC_VehicleSpeed_mph_Inproc/1 -> UnitConverter1061/1
  UnitConverter1061/1 -> VOUTP_VehicleSpeed_mph/1  "VOUTP_VehicleSpeed_mph"
  VVMC_VehicleSpeed_kph/1 -> VVMC_VehicleSpeed_kph_Inproc/1  "VVMC_VehicleSpeed_kph"
  VVMC_VehicleSpeed_kph_Inproc/1 -> UnitConverter1062/1
  UnitConverter1062/1 -> VOUTP_VehicleSpeed_kph/1  "VOUTP_VehicleSpeed_kph"
  VVMC_MeterIndSpeed_raw32/1 -> VVMC_MeterIndSpeed_raw32_Inproc/1  "VVMC_MeterIndSpeed_raw32"
  VVMC_MeterIndSpeed_raw32_Inproc/1 -> UnitConverter1063/1
  UnitConverter1063/1 -> VOUTP_MeterIndSpeed_raw32/1  "VOUTP_MeterIndSpeed_raw32"
  VVMC_VMCAEBCtrlAvail_flg/1 -> VVMC_VMCAEBCtrlAvail_flg_Inproc/1  "VVMC_VMCAEBCtrlAvail_flg"
  VVMC_VMCAEBCtrlAvail_flg_Inproc/1 -> UnitConverter1064/1
  UnitConverter1064/1 -> VOUTP_VMCAEBCtrlAvail_flg/1  "VOUTP_VMCAEBCtrlAvail_flg"
  VVMC_VMCACCCtrlAvail_flg/1 -> VVMC_VMCACCCtrlAvail_flg_Inproc/1  "VVMC_VMCACCCtrlAvail_flg"
  VVMC_VMCACCCtrlAvail_flg_Inproc/1 -> UnitConverter1065/1
  UnitConverter1065/1 -> VOUTP_VMCACCCtrlAvail_flg/1  "VOUTP_VMCACCCtrlAvail_flg"
  VVMC_VMCCCCtrlAvail_flg/1 -> VVMC_VMCCCCtrlAvail_flg_Inproc/1  "VVMC_VMCCCCtrlAvail_flg"
  VVMC_VMCCCCtrlAvail_flg_Inproc/1 -> UnitConverter1066/1
  UnitConverter1066/1 -> VOUTP_VMCCCCtrlAvail_flg/1  "VOUTP_VMCCCCtrlAvail_flg"
  VVMC_VMCMSACtrlAvail_flg/1 -> VVMC_VMCMSACtrlAvail_flg_Inproc/1  "VVMC_VMCMSACtrlAvail_flg"
  VVMC_VMCMSACtrlAvail_flg_Inproc/1 -> UnitConverter1067/1
  UnitConverter1067/1 -> VOUTP_VMCMSACtrlAvail_flg/1  "VOUTP_VMCMSACtrlAvail_flg"
  VVMC_FeatArbitrSta_enum/1 -> VVMC_FeatArbitrSta_enum_Inproc/1  "VVMC_FeatArbitrSta_enum"
  VVMC_FeatArbitrSta_enum_Inproc/1 -> UnitConverter1068/1
  UnitConverter1068/1 -> VOUTP_FeatArbitrSta_enum/1  "VOUTP_FeatArbitrSta_enum"
  VVMC_FeatReqSpd_kph/1 -> VVMC_FeatReqSpd_kph_Inproc/1  "VVMC_FeatReqSpd_kph"
  VVMC_FeatReqSpd_kph_Inproc/1 -> UnitConverter1069/1
  UnitConverter1069/1 -> VOUTP_FeatReqSpd_kph/1  "VOUTP_FeatReqSpd_kph"
  VVMC_JerkPCT_pct/1 -> VVMC_JerkPCT_pct_Inproc/1  "VVMC_JerkPCT_pct"
  VVMC_JerkPCT_pct_Inproc/1 -> UnitConverter1070/1
  UnitConverter1070/1 -> VOUTP_JerkPCT_pct/1  "VOUTP_JerkPCT_pct"
  VVMC_LimitPCT_pct/1 -> VVMC_LimitPCT_pct_Inproc/1  "VVMC_LimitPCT_pct"
  VVMC_LimitPCT_pct_Inproc/1 -> UnitConverter1071/1
  UnitConverter1071/1 -> VOUTP_LimitPCT_pct/1  "VOUTP_LimitPCT_pct"
  VVMC_FrontRearSlipRatioCtrl_flg/1 -> VVMC_FrontRearSlipRatioCtrl_flg_Inproc/1  "VVMC_FrontRearSlipRatioCtrl_flg"
  VVMC_FrontRearSlipRatioCtrl_flg_Inproc/1 -> UnitConverter1072/1
  UnitConverter1072/1 -> VOUTP_FrontRearSlipRatioCtrl_flg/1  "VOUTP_FrontRearSlipRatioCtrl_flg"
  VVMC_RearWhlSlipRatioCtrl_flg/1 -> VVMC_RearWhlSlipRatioCtrl_flg_Inproc/1  "VVMC_RearWhlSlipRatioCtrl_flg"
  VVMC_RearWhlSlipRatioCtrl_flg_Inproc/1 -> UnitConverter1073/1
  UnitConverter1073/1 -> VOUTP_RearWhlSlipRatioCtrl_flg/1  "VOUTP_RearWhlSlipRatioCtrl_flg"
  VVMC_SingleWhlSlipRatioCtrl_flg/1 -> VVMC_SingleWhlSlipRatioCtrl_flg_Inproc/1  "VVMC_SingleWhlSlipRatioCtrl_flg"
  VVMC_SingleWhlSlipRatioCtrl_flg_Inproc/1 -> UnitConverter1074/1
  UnitConverter1074/1 -> VOUTP_SingleWhlSlipRatioCtrl_flg/1  "VOUTP_SingleWhlSlipRatioCtrl_flg"
  VVMC_LatAccCtrl_flg/1 -> VVMC_LatAccCtrl_flg_Inproc/1  "VVMC_LatAccCtrl_flg"
  VVMC_LatAccCtrl_flg_Inproc/1 -> UnitConverter1075/1
  UnitConverter1075/1 -> VOUTP_LatAccCtrl_flg/1  "VOUTP_LatAccCtrl_flg"
  VVMC_SafetyCtrl_flg/1 -> VVMC_SafetyCtrl_flg_Inproc/1  "VVMC_SafetyCtrl_flg"
  VVMC_SafetyCtrl_flg_Inproc/1 -> UnitConverter1076/1
  UnitConverter1076/1 -> VOUTP_SafetyCtrl_flg/1  "VOUTP_SafetyCtrl_flg"
  VVMC_SPD2ACCAct_flg/1 -> VVMC_SPD2ACCAct_flg_Inproc/1  "VVMC_SPD2ACCAct_flg"
  VVMC_SPD2ACCAct_flg_Inproc/1 -> UnitConverter1077/1
  UnitConverter1077/1 -> VOUTP_SPD2ACCAct_flg/1  "VOUTP_SPD2ACCAct_flg"
  VVMC_AccCalcuPID_mps2/1 -> VVMC_AccCalcuPID_mps2_Inproc/1  "VVMC_AccCalcuPID_mps2"
  VVMC_AccCalcuPID_mps2_Inproc/1 -> UnitConverter1078/1
  UnitConverter1078/1 -> VOUTP_AccCalcuPID_mps2/1  "VOUTP_AccCalcuPID_mps2"
  VVMC_ISOAccLimit_mps2/1 -> VVMC_ISOAccLimit_mps2_Inproc/1  "VVMC_ISOAccLimit_mps2"
  VVMC_ISOAccLimit_mps2_Inproc/1 -> UnitConverter1079/1
  UnitConverter1079/1 -> VOUTP_ISOAccLimit_mps2/1  "VOUTP_ISOAccLimit_mps2"
  VVMC_ISODecLimit_mps2/1 -> VVMC_ISODecLimit_mps2_Inproc/1  "VVMC_ISODecLimit_mps2"
  VVMC_ISODecLimit_mps2_Inproc/1 -> UnitConverter1080/1
  UnitConverter1080/1 -> VOUTP_ISODecLimit_mps2/1  "VOUTP_ISODecLimit_mps2"
  VVMC_ISOJerkLimit_mps3/1 -> VVMC_ISOJerkLimit_mps3_Inproc/1  "VVMC_ISOJerkLimit_mps3"
  VVMC_ISOJerkLimit_mps3_Inproc/1 -> UnitConverter1081/1
  UnitConverter1081/1 -> VOUTP_ISOJerkLimit_mps3/1  "VOUTP_ISOJerkLimit_mps3"
  VVMC_ACCRequiredAccel_mps2/1 -> VVMC_ACCRequiredAccel_mps2_Inproc/1  "VVMC_ACCRequiredAccel_mps2"
  VVMC_ACCRequiredAccel_mps2_Inproc/1 -> UnitConverter1082/1
  UnitConverter1082/1 -> VOUTP_ACCRequiredAccel_mps2/1  "VOUTP_ACCRequiredAccel_mps2"
  VVMC_DISCReqAcc_mps2/1 -> VVMC_DISCReqAcc_mps2_Inproc/1  "VVMC_DISCReqAcc_mps2"
  VVMC_DISCReqAcc_mps2_Inproc/1 -> UnitConverter1083/1
  UnitConverter1083/1 -> VOUTP_DISCReqAcc_mps2/1  "VOUTP_DISCReqAcc_mps2"
  VVMC_FeatArbitrFinal_enum/1 -> VVMC_FeatArbitrFinal_enum_Inproc/1  "VVMC_FeatArbitrFinal_enum"
  VVMC_FeatArbitrFinal_enum_Inproc/1 -> UnitConverter1084/1
  UnitConverter1084/1 -> VOUTP_FeatArbitrFinal_enum/1  "VOUTP_FeatArbitrFinal_enum"
  VVMC_ActACCRequiredAccel_mps2/1 -> VVMC_ActACCRequiredAccel_mps2_Inproc/1  "VVMC_ActACCRequiredAccel_mps2"
  VVMC_ActACCRequiredAccel_mps2_Inproc/1 -> UnitConverter1085/1
  UnitConverter1085/1 -> VOUTP_ActACCRequiredAccel_mps2/1  "VOUTP_ActACCRequiredAccel_mps2"
  VVMC_LateralCtrl_flg/1 -> VVMC_LateralCtrl_flg_Inproc/1  "VVMC_LateralCtrl_flg"
  VVMC_LateralCtrl_flg_Inproc/1 -> UnitConverter1086/1
  UnitConverter1086/1 -> VOUTP_LateralCtrl_flg/1  "VOUTP_LateralCtrl_flg"
  VVMC_ADASLKASta_enum/1 -> VVMC_ADASLKASta_enum_Inproc/1  "VVMC_ADASLKASta_enum"
  VVMC_ADASLKASta_enum_Inproc/1 -> UnitConverter1087/1
  UnitConverter1087/1 -> VOUTP_ADASLKASta_enum/1  "VOUTP_ADASLKASta_enum"
  VVMC_LKAStrToqReq_Nm/1 -> VVMC_LKAStrToqReq_Nm_Inproc/1  "VVMC_LKAStrToqReq_Nm"
  VVMC_LKAStrToqReq_Nm_Inproc/1 -> UnitConverter1088/1
  UnitConverter1088/1 -> VOUTP_LKAStrToqReq_Nm/1  "VOUTP_LKAStrToqReq_Nm"
  VVMC_LKATOIFault_flg/1 -> VVMC_LKATOIFault_flg_Inproc/1  "VVMC_LKATOIFault_flg"
  VVMC_LKATOIFault_flg_Inproc/1 -> UnitConverter1089/1
  UnitConverter1089/1 -> VOUTP_LKATOIFault_flg/1  "VOUTP_LKATOIFault_flg"
  VVMC_LKATOIAct_enum/1 -> VVMC_LKATOIAct_enum_Inproc/1  "VVMC_LKATOIAct_enum"
  VVMC_LKATOIAct_enum_Inproc/1 -> UnitConverter1090/1
  UnitConverter1090/1 -> VOUTP_LKATOIAct_enum/1  "VOUTP_LKATOIAct_enum"
  VVMC_ADASAEBReq_enum/1 -> VVMC_ADASAEBReq_enum_Inproc/1  "VVMC_ADASAEBReq_enum"
  VVMC_ADASAEBReq_enum_Inproc/1 -> UnitConverter1091/1
  UnitConverter1091/1 -> VOUTP_ADASAEBReq_enum/1  "VOUTP_ADASAEBReq_enum"
  VVMC_ADASFaultSta_flg/1 -> VVMC_ADASFaultSta_flg_Inproc/1  "VVMC_ADASFaultSta_flg"
  VVMC_ADASFaultSta_flg_Inproc/1 -> UnitConverter1092/1
  UnitConverter1092/1 -> VOUTP_ADASFaultSta_flg/1  "VOUTP_ADASFaultSta_flg"
  VVMC_AEBVehHoldReq_flg/1 -> VVMC_AEBVehHoldReq_flg_Inproc/1  "VVMC_AEBVehHoldReq_flg"
  VVMC_AEBVehHoldReq_flg_Inproc/1 -> UnitConverter1093/1
  UnitConverter1093/1 -> VOUTP_AEBVehHoldReq_flg/1  "VOUTP_AEBVehHoldReq_flg"
  VVMC_ACCVehHoldReq_flg/1 -> VVMC_ACCVehHoldReq_flg_Inproc/1  "VVMC_ACCVehHoldReq_flg"
  VVMC_ACCVehHoldReq_flg_Inproc/1 -> UnitConverter1094/1
  UnitConverter1094/1 -> VOUTP_ACCVehHoldReq_flg/1  "VOUTP_ACCVehHoldReq_flg"
  VVMC_ADASDBSReq_enum/1 -> VVMC_ADASDBSReq_enum_Inproc/1  "VVMC_ADASDBSReq_enum"
  VVMC_ADASDBSReq_enum_Inproc/1 -> UnitConverter1095/1
  UnitConverter1095/1 -> VOUTP_ADASDBSReq_enum/1  "VOUTP_ADASDBSReq_enum"
  VVMC_ADASACCSta_enum/1 -> VVMC_ADASACCSta_enum_Inproc/1  "VVMC_ADASACCSta_enum"
  VVMC_ADASACCSta_enum_Inproc/1 -> UnitConverter1096/1
  UnitConverter1096/1 -> VOUTP_ADASACCSta_enum/1  "VOUTP_ADASACCSta_enum"
  VVMC_ACCObjDist_m/1 -> VVMC_ACCObjDist_m_Inproc/1  "VVMC_ACCObjDist_m"
  VVMC_ACCObjDist_m_Inproc/1 -> UnitConverter1097/1
  UnitConverter1097/1 -> VOUTP_ACCObjDist_m/1  "VOUTP_ACCObjDist_m"
  VVMC_ACCObjRelSpd_mps/1 -> VVMC_ACCObjRelSpd_mps_Inproc/1  "VVMC_ACCObjRelSpd_mps"
  VVMC_ACCObjRelSpd_mps_Inproc/1 -> UnitConverter1098/1
  UnitConverter1098/1 -> VOUTP_ACCObjRelSpd_mps/1  "VOUTP_ACCObjRelSpd_mps"
  VVMC_TimeGapLevel_enum/1 -> VVMC_TimeGapLevel_enum_Inproc/1  "VVMC_TimeGapLevel_enum"
  VVMC_TimeGapLevel_enum_Inproc/1 -> UnitConverter1099/1
  UnitConverter1099/1 -> VOUTP_TimeGapLevel_enum/1  "VOUTP_TimeGapLevel_enum"
  VVMC_ACCJerkUpperLimit_mps3/1 -> VVMC_ACCJerkUpperLimit_mps3_Inproc/1  "VVMC_ACCJerkUpperLimit_mps3"
  VVMC_ACCJerkUpperLimit_mps3_Inproc/1 -> UnitConverter1100/1
  UnitConverter1100/1 -> VOUTP_ACCJerkUpperLimit_mps3/1  "VOUTP_ACCJerkUpperLimit_mps3"
  VVMC_ACCComfortBandUpper_mps2/1 -> VVMC_ACCComfortBandUpper_mps2_Inproc/1  "VVMC_ACCComfortBandUpper_mps2"
  VVMC_ACCComfortBandUpper_mps2_Inproc/1 -> UnitConverter1101/1
  UnitConverter1101/1 -> VOUTP_ACCComfortBandUpper_mps2/1  "VOUTP_ACCComfortBandUpper_mps2"
  VVMC_ACCJerkLowerLimit_mps3/1 -> VVMC_ACCJerkLowerLimit_mps3_Inproc/1  "VVMC_ACCJerkLowerLimit_mps3"
  VVMC_ACCJerkLowerLimit_mps3_Inproc/1 -> UnitConverter1102/1
  UnitConverter1102/1 -> VOUTP_ACCJerkLowerLimit_mps3/1  "VOUTP_ACCJerkLowerLimit_mps3"
  VVMC_ACCComfortBandLower_mps2/1 -> VVMC_ACCComfortBandLower_mps2_Inproc/1  "VVMC_ACCComfortBandLower_mps2"
  VVMC_ACCComfortBandLower_mps2_Inproc/1 -> UnitConverter1103/1
  UnitConverter1103/1 -> VOUTP_ACCComfortBandLower_mps2/1  "VOUTP_ACCComfortBandLower_mps2"
  VVMC_ADASVehSpdLim_raw32/1 -> VVMC_ADASVehSpdLim_raw32_Inproc/1  "VVMC_ADASVehSpdLim_raw32"
  VVMC_ADASVehSpdLim_raw32_Inproc/1 -> UnitConverter1104/1
  UnitConverter1104/1 -> VOUTP_ADASVehSpdLim_raw32/1  "VOUTP_ADASVehSpdLim_raw32"
  VVMC_ADASShftPosnReqA_flg/1 -> VVMC_ADASShftPosnReqA_flg_Inproc/1  "VVMC_ADASShftPosnReqA_flg"
  VVMC_ADASShftPosnReqA_flg_Inproc/1 -> UnitConverter1105/1
  UnitConverter1105/1 -> VOUTP_ADASShftPosnReqA_flg/1  "VOUTP_ADASShftPosnReqA_flg"
  VVMC_ADASShftPosnReq_enum/1 -> VVMC_ADASShftPosnReq_enum_Inproc/1  "VVMC_ADASShftPosnReq_enum"
  VVMC_ADASShftPosnReq_enum_Inproc/1 -> UnitConverter1106/1
  UnitConverter1106/1 -> VOUTP_ADASShftPosnReq_enum/1  "VOUTP_ADASShftPosnReq_enum"
  VVMC_ADASForceIdle_flg/1 -> VVMC_ADASForceIdle_flg_Inproc/1  "VVMC_ADASForceIdle_flg"
  VVMC_ADASForceIdle_flg_Inproc/1 -> UnitConverter1107/1
  UnitConverter1107/1 -> VOUTP_ADASForceIdle_flg/1  "VOUTP_ADASForceIdle_flg"
  VVMC_HazardWarningReq_flg/1 -> VVMC_HazardWarningReq_flg_Inproc/1  "VVMC_HazardWarningReq_flg"
  VVMC_HazardWarningReq_flg_Inproc/1 -> UnitConverter1108/1
  UnitConverter1108/1 -> VOUTP_HazardWarningReq_flg/1  "VOUTP_HazardWarningReq_flg"
  VVMC_RightTurnLightReq_flg/1 -> VVMC_RightTurnLightReq_flg_Inproc/1  "VVMC_RightTurnLightReq_flg"
  VVMC_RightTurnLightReq_flg_Inproc/1 -> UnitConverter1109/1
  UnitConverter1109/1 -> VOUTP_RightTurnLightReq_flg/1  "VOUTP_RightTurnLightReq_flg"
  VVMC_LeftTurnLightReq_flg/1 -> VVMC_LeftTurnLightReq_flg_Inproc/1  "VVMC_LeftTurnLightReq_flg"
  VVMC_LeftTurnLightReq_flg_Inproc/1 -> UnitConverter1110/1
  UnitConverter1110/1 -> VOUTP_LeftTurnLightReq_flg/1  "VOUTP_LeftTurnLightReq_flg"
  VVMC_ADASFCWSta_enum/1 -> VVMC_ADASFCWSta_enum_Inproc/1  "VVMC_ADASFCWSta_enum"
  VVMC_ADASFCWSta_enum_Inproc/1 -> UnitConverter1111/1
  UnitConverter1111/1 -> VOUTP_ADASFCWSta_enum/1  "VOUTP_ADASFCWSta_enum"
  VVMC_ADASLDWSta_enum/1 -> VVMC_ADASLDWSta_enum_Inproc/1  "VVMC_ADASLDWSta_enum"
  VVMC_ADASLDWSta_enum_Inproc/1 -> UnitConverter1112/1
  UnitConverter1112/1 -> VOUTP_ADASLDWSta_enum/1  "VOUTP_ADASLDWSta_enum"
  VVMC_ADASFltWrnReq_flg/1 -> VVMC_ADASFltWrnReq_flg_Inproc/1  "VVMC_ADASFltWrnReq_flg"
  VVMC_ADASFltWrnReq_flg_Inproc/1 -> UnitConverter1113/1
  UnitConverter1113/1 -> VOUTP_ADASFltWrnReq_flg/1  "VOUTP_ADASFltWrnReq_flg"
  VVMC_ACCObjDstLvl_enum/1 -> VVMC_ACCObjDstLvl_enum_Inproc/1  "VVMC_ACCObjDstLvl_enum"
  VVMC_ACCObjDstLvl_enum_Inproc/1 -> UnitConverter1114/1
  UnitConverter1114/1 -> VOUTP_ACCObjDstLvl_enum/1  "VOUTP_ACCObjDstLvl_enum"
  VVMC_ForceLowBeam_enum/1 -> VVMC_ForceLowBeam_enum_Inproc/1  "VVMC_ForceLowBeam_enum"
  VVMC_ForceLowBeam_enum_Inproc/1 -> UnitConverter1115/1
  UnitConverter1115/1 -> VOUTP_ForceLowBeam_enum/1  "VOUTP_ForceLowBeam_enum"
  VVMC_ACCTakeoverReq_flg/1 -> VVMC_ACCTakeoverReq_flg_Inproc/1  "VVMC_ACCTakeoverReq_flg"
  VVMC_ACCTakeoverReq_flg_Inproc/1 -> UnitConverter1116/1
  UnitConverter1116/1 -> VOUTP_ACCTakeoverReq_flg/1  "VOUTP_ACCTakeoverReq_flg"
  VVMC_ADASWarningMsg_enum/1 -> VVMC_ADASWarningMsg_enum_Inproc/1  "VVMC_ADASWarningMsg_enum"
  VVMC_ADASWarningMsg_enum_Inproc/1 -> UnitConverter1117/1
  UnitConverter1117/1 -> VOUTP_ADASWarningMsg_enum/1  "VOUTP_ADASWarningMsg_enum"
  VVMC_ADASCAMSpdLim_enum/1 -> VVMC_ADASCAMSpdLim_enum_Inproc/1  "VVMC_ADASCAMSpdLim_enum"
  VVMC_ADASCAMSpdLim_enum_Inproc/1 -> UnitConverter1118/1
  UnitConverter1118/1 -> VOUTP_ADASCAMSpdLim_enum/1  "VOUTP_ADASCAMSpdLim_enum"
  VVMC_TargetType_enum/1 -> VVMC_TargetType_enum_Inproc/1  "VVMC_TargetType_enum"
  VVMC_TargetType_enum_Inproc/1 -> UnitConverter1119/1
  UnitConverter1119/1 -> VOUTP_TargetType_enum/1  "VOUTP_TargetType_enum"
  VVMC_ADASSLIFSpdLim_enum/1 -> VVMC_ADASSLIFSpdLim_enum_Inproc/1  "VVMC_ADASSLIFSpdLim_enum"
  VVMC_ADASSLIFSpdLim_enum_Inproc/1 -> UnitConverter1120/1
  UnitConverter1120/1 -> VOUTP_ADASSLIFSpdLim_enum/1  "VOUTP_ADASSLIFSpdLim_enum"
  VVMC_LKAHODDisplayWarning_flg/1 -> VVMC_LKAHODDisplayWarning_flg_Inproc/1  "VVMC_LKAHODDisplayWarning_flg"
  VVMC_LKAHODDisplayWarning_flg_Inproc/1 -> UnitConverter1121/1
  UnitConverter1121/1 -> VOUTP_LKAHODDisplayWarning_flg/1  "VOUTP_LKAHODDisplayWarning_flg"
  VVMC_LKAHODSoundWarning_flg/1 -> VVMC_LKAHODSoundWarning_flg_Inproc/1  "VVMC_LKAHODSoundWarning_flg"
  VVMC_LKAHODSoundWarning_flg_Inproc/1 -> UnitConverter1122/1
  UnitConverter1122/1 -> VOUTP_LKAHODSoundWarning_flg/1  "VOUTP_LKAHODSoundWarning_flg"
  VVMC_ADASLFCSta_enum/1 -> VVMC_ADASLFCSta_enum_Inproc/1  "VVMC_ADASLFCSta_enum"
  VVMC_ADASLFCSta_enum_Inproc/1 -> UnitConverter1123/1
  UnitConverter1123/1 -> VOUTP_ADASLFCSta_enum/1  "VOUTP_ADASLFCSta_enum"
  VVMC_ADASLaneModeL_enum/1 -> VVMC_ADASLaneModeL_enum_Inproc/1  "VVMC_ADASLaneModeL_enum"
  VVMC_ADASLaneModeL_enum_Inproc/1 -> UnitConverter1124/1
  UnitConverter1124/1 -> VOUTP_ADASLaneModeL_enum/1  "VOUTP_ADASLaneModeL_enum"
  VVMC_ADASLaneModeR_enum/1 -> VVMC_ADASLaneModeR_enum_Inproc/1  "VVMC_ADASLaneModeR_enum"
  VVMC_ADASLaneModeR_enum_Inproc/1 -> UnitConverter1125/1
  UnitConverter1125/1 -> VOUTP_ADASLaneModeR_enum/1  "VOUTP_ADASLaneModeR_enum"
  VVMC_ADASSLIFSta_enum/1 -> VVMC_ADASSLIFSta_enum_Inproc/1  "VVMC_ADASSLIFSta_enum"
  VVMC_ADASSLIFSta_enum_Inproc/1 -> UnitConverter1126/1
  UnitConverter1126/1 -> VOUTP_ADASSLIFSta_enum/1  "VOUTP_ADASSLIFSta_enum"
  VVMC_ADASISASta_enum/1 -> VVMC_ADASISASta_enum_Inproc/1  "VVMC_ADASISASta_enum"
  VVMC_ADASISASta_enum_Inproc/1 -> UnitConverter1127/1
  UnitConverter1127/1 -> VOUTP_ADASISASta_enum/1  "VOUTP_ADASISASta_enum"
  VVMC_ADASLDWMute_flg/1 -> VVMC_ADASLDWMute_flg_Inproc/1  "VVMC_ADASLDWMute_flg"
  VVMC_ADASLDWMute_flg_Inproc/1 -> UnitConverter1128/1
  UnitConverter1128/1 -> VOUTP_ADASLDWMute_flg/1  "VOUTP_ADASLDWMute_flg"
  VVMC_ADASFCWMute_flg/1 -> VVMC_ADASFCWMute_flg_Inproc/1  "VVMC_ADASFCWMute_flg"
  VVMC_ADASFCWMute_flg_Inproc/1 -> UnitConverter1129/1
  UnitConverter1129/1 -> VOUTP_ADASFCWMute_flg/1  "VOUTP_ADASFCWMute_flg"
  VVMC_ADASLFCHandsOffWarning_enum/1 -> VVMC_ADASLFCHandsOffWarning_enum_Inproc/1  "VVMC_ADASLFCHandsOffWarning_enum"
  VVMC_ADASLFCHandsOffWarning_enum_Inproc/1 -> UnitConverter1130/1
  UnitConverter1130/1 -> VOUTP_ADASLFCHandsOffWarning_enum/1  "VOUTP_ADASLFCHandsOffWarning_enum"
  VVMC_LVDADisabled_flg/1 -> VVMC_LVDADisabled_flg_Inproc/1  "VVMC_LVDADisabled_flg"
  VVMC_LVDADisabled_flg_Inproc/1 -> UnitConverter1131/1
  UnitConverter1131/1 -> VOUTP_LVDADisabled_flg/1  "VOUTP_LVDADisabled_flg"
  VVMC_LVDAMuteSta_enum/1 -> VVMC_LVDAMuteSta_enum_Inproc/1  "VVMC_LVDAMuteSta_enum"
  VVMC_LVDAMuteSta_enum_Inproc/1 -> UnitConverter1132/1
  UnitConverter1132/1 -> VOUTP_LVDAMuteSta_enum/1  "VOUTP_LVDAMuteSta_enum"
  VVMC_LVDAFailinfo_flg/1 -> VVMC_LVDAFailinfo_flg_Inproc/1  "VVMC_LVDAFailinfo_flg"
  VVMC_LVDAFailinfo_flg_Inproc/1 -> UnitConverter1133/1
  UnitConverter1133/1 -> VOUTP_LVDAFailinfo_flg/1  "VOUTP_LVDAFailinfo_flg"
  VVMC_LVDAWarning_flg/1 -> VVMC_LVDAWarning_flg_Inproc/1  "VVMC_LVDAWarning_flg"
  VVMC_LVDAWarning_flg_Inproc/1 -> UnitConverter1134/1
  UnitConverter1134/1 -> VOUTP_LVDAWarning_flg/1  "VOUTP_LVDAWarning_flg"
  VVMC_LVDAACCStatusInformation_flg/1 -> VVMC_LVDAACCStatusInformation_flg_Inproc/1  "VVMC_LVDAACCStatusInformation_flg"
  VVMC_LVDAACCStatusInformation_flg_Inproc/1 -> UnitConverter1135/1
  UnitConverter1135/1 -> VOUTP_LVDAACCStatusInformation_flg/1  "VOUTP_LVDAACCStatusInformation_flg"
  VVMC_ADASLFCWarnSound_enum/1 -> VVMC_ADASLFCWarnSound_enum_Inproc/1  "VVMC_ADASLFCWarnSound_enum"
  VVMC_ADASLFCWarnSound_enum_Inproc/1 -> UnitConverter1136/1
  UnitConverter1136/1 -> VOUTP_ADASLFCWarnSound_enum/1  "VOUTP_ADASLFCWarnSound_enum"
  VVMC_FCMACCmode_enum/1 -> VVMC_FCMACCmode_enum_Inproc/1  "VVMC_FCMACCmode_enum"
  VVMC_FCMACCmode_enum_Inproc/1 -> UnitConverter1137/1
  UnitConverter1137/1 -> VOUTP_FCMACCmode_enum/1  "VOUTP_FCMACCmode_enum"
  VVMC_ADASLanetypeR_enum/1 -> VVMC_ADASLanetypeR_enum_Inproc/1  "VVMC_ADASLanetypeR_enum"
  VVMC_ADASLanetypeR_enum_Inproc/1 -> UnitConverter1138/1
  UnitConverter1138/1 -> VOUTP_ADASLanetypeR_enum/1  "VOUTP_ADASLanetypeR_enum"
  VVMC_ADASLanetypeL_enum/1 -> VVMC_ADASLanetypeL_enum_Inproc/1  "VVMC_ADASLanetypeL_enum"
  VVMC_ADASLanetypeL_enum_Inproc/1 -> UnitConverter1139/1
  UnitConverter1139/1 -> VOUTP_ADASLanetypeL_enum/1  "VOUTP_ADASLanetypeL_enum"
  VVMC_ADASLanecurveL_raw32/1 -> VVMC_ADASLanecurveL_raw32_Inproc/1  "VVMC_ADASLanecurveL_raw32"
  VVMC_ADASLanecurveL_raw32_Inproc/1 -> UnitConverter1140/1
  UnitConverter1140/1 -> VOUTP_ADASLanecurveL_raw32/1  "VOUTP_ADASLanecurveL_raw32"
  VVMC_ADASLanecurveR_raw32/1 -> VVMC_ADASLanecurveR_raw32_Inproc/1  "VVMC_ADASLanecurveR_raw32"
  VVMC_ADASLanecurveR_raw32_Inproc/1 -> UnitConverter1141/1
  UnitConverter1141/1 -> VOUTP_ADASLanecurveR_raw32/1  "VOUTP_ADASLanecurveR_raw32"
  VVMC_ADASAEBSta_enum/1 -> VVMC_ADASAEBSta_enum_Inproc/1  "VVMC_ADASAEBSta_enum"
  VVMC_ADASAEBSta_enum_Inproc/1 -> UnitConverter1142/1
  UnitConverter1142/1 -> VOUTP_ADASAEBSta_enum/1  "VOUTP_ADASAEBSta_enum"
  VVMC_FCMLDWRequest_enum/1 -> VVMC_FCMLDWRequest_enum_Inproc/1  "VVMC_FCMLDWRequest_enum"
  VVMC_FCMLDWRequest_enum_Inproc/1 -> UnitConverter1143/1
  UnitConverter1143/1 -> VOUTP_FCMLDWRequest_enum/1  "VOUTP_FCMLDWRequest_enum"
  VVMC_FCMLDWFault_flg/1 -> VVMC_FCMLDWFault_flg_Inproc/1  "VVMC_FCMLDWFault_flg"
  VVMC_FCMLDWFault_flg_Inproc/1 -> UnitConverter1144/1
  UnitConverter1144/1 -> VOUTP_FCMLDWFault_flg/1  "VOUTP_FCMLDWFault_flg"
  VVMC_ACCCtrlAvail_flg/1 -> VVMC_ACCCtrlAvail_flg_Inproc/1  "VVMC_ACCCtrlAvail_flg"
  VVMC_ACCCtrlAvail_flg_Inproc/1 -> UnitConverter1145/1
  UnitConverter1145/1 -> VOUTP_ACCCtrlAvail_flg/1  "VOUTP_ACCCtrlAvail_flg"
  VVMC_ACCPedalOvrd_flg/1 -> VVMC_ACCPedalOvrd_flg_Inproc/1  "VVMC_ACCPedalOvrd_flg"
  VVMC_ACCPedalOvrd_flg_Inproc/1 -> UnitConverter1146/1
  UnitConverter1146/1 -> VOUTP_ACCPedalOvrd_flg/1  "VOUTP_ACCPedalOvrd_flg"
  VVMC_TimeGapCalcu_s/1 -> VVMC_TimeGapCalcu_s_Inproc/1  "VVMC_TimeGapCalcu_s"
  VVMC_TimeGapCalcu_s_Inproc/1 -> UnitConverter1147/1
  UnitConverter1147/1 -> VOUTP_TimeGapCalcu_s/1  "VOUTP_TimeGapCalcu_s"
  VVMC_CCCtrlSta_enum/1 -> VVMC_CCCtrlSta_enum_Inproc/1  "VVMC_CCCtrlSta_enum"
  VVMC_CCCtrlSta_enum_Inproc/1 -> UnitConverter1148/1
  UnitConverter1148/1 -> VOUTP_CCCtrlSta_enum/1  "VOUTP_CCCtrlSta_enum"
  VVMC_MSACtrlSta_enum/1 -> VVMC_MSACtrlSta_enum_Inproc/1  "VVMC_MSACtrlSta_enum"
  VVMC_MSACtrlSta_enum_Inproc/1 -> UnitConverter1149/1
  UnitConverter1149/1 -> VOUTP_MSACtrlSta_enum/1  "VOUTP_MSACtrlSta_enum"
  VVMC_APSCtrlAvail_flg/1 -> VVMC_APSCtrlAvail_flg_Inproc/1  "VVMC_APSCtrlAvail_flg"
  VVMC_APSCtrlAvail_flg_Inproc/1 -> UnitConverter1150/1
  UnitConverter1150/1 -> VOUTP_APSCtrlAvail_flg/1  "VOUTP_APSCtrlAvail_flg"
  VVMC_APSActive_flg/1 -> VVMC_APSActive_flg_Inproc/1  "VVMC_APSActive_flg"
  VVMC_APSActive_flg_Inproc/1 -> UnitConverter1151/1
  UnitConverter1151/1 -> VOUTP_APSActive_flg/1  "VOUTP_APSActive_flg"
  VVMC_APSStaSys_enum/1 -> VVMC_APSStaSys_enum_Inproc/1  "VVMC_APSStaSys_enum"
  VVMC_APSStaSys_enum_Inproc/1 -> UnitConverter1152/1
  UnitConverter1152/1 -> VOUTP_APSStaSys_enum/1  "VOUTP_APSStaSys_enum"
  VVMC_APSDecReqA_flg/1 -> VVMC_APSDecReqA_flg_Inproc/1  "VVMC_APSDecReqA_flg"
  VVMC_APSDecReqA_flg_Inproc/1 -> UnitConverter1153/1
  UnitConverter1153/1 -> VOUTP_APSDecReqA_flg/1  "VOUTP_APSDecReqA_flg"
  VVMC_APSDecReq_mps2/1 -> VVMC_APSDecReq_mps2_Inproc/1  "VVMC_APSDecReq_mps2"
  VVMC_APSDecReq_mps2_Inproc/1 -> UnitConverter1154/1
  UnitConverter1154/1 -> VOUTP_APSDecReq_mps2/1  "VOUTP_APSDecReq_mps2"
  VVMC_APSReq_enum/1 -> VVMC_APSReq_enum_Inproc/1  "VVMC_APSReq_enum"
  VVMC_APSReq_enum_Inproc/1 -> UnitConverter1155/1
  UnitConverter1155/1 -> VOUTP_APSReq_enum/1  "VOUTP_APSReq_enum"
  VVMC_LongAcc_Gps/1 -> VVMC_LongAcc_Gps_Inproc/1  "VVMC_LongAcc_Gps"
  VVMC_LongAcc_Gps_Inproc/1 -> UnitConverter1156/1
  UnitConverter1156/1 -> VOUTP_LongAcc_Gps/1  "VOUTP_LongAcc_Gps"
  VVMC_CCMSASpdWar_flg/1 -> VVMC_CCMSASpdWar_flg_Inproc/1  "VVMC_CCMSASpdWar_flg"
  VVMC_CCMSASpdWar_flg_Inproc/1 -> UnitConverter1157/1
  UnitConverter1157/1 -> VOUTP_CCMSASpdWar_flg/1  "VOUTP_CCMSASpdWar_flg"
  VVMC_IMUEnaCmd_flg/1 -> VVMC_IMUEnaCmd_flg_Inproc/1  "VVMC_IMUEnaCmd_flg"
  VVMC_IMUEnaCmd_flg_Inproc/1 -> UnitConverter1158/1
  UnitConverter1158/1 -> VOUTP_IMUEnaCmd_flg/1  "VOUTP_IMUEnaCmd_flg"
  VVMC_ActStESCYaw_Dps/1 -> VVMC_ActStESCYaw_Dps_Inproc/1  "VVMC_ActStESCYaw_Dps"
  VVMC_ActStESCYaw_Dps_Inproc/1 -> UnitConverter1159/1
  UnitConverter1159/1 -> VOUTP_ActStESCYaw_Dps/1  "VOUTP_ActStESCYaw_Dps"
  VVMC_CAASCtrlAvail_flg/1 -> VVMC_CAASCtrlAvail_flg_Inproc/1  "VVMC_CAASCtrlAvail_flg"
  VVMC_CAASCtrlAvail_flg_Inproc/1 -> UnitConverter1160/1
  UnitConverter1160/1 -> VOUTP_CAASCtrlAvail_flg/1  "VOUTP_CAASCtrlAvail_flg"
  VVMC_CAASActive_flg/1 -> VVMC_CAASActive_flg_Inproc/1  "VVMC_CAASActive_flg"
  VVMC_CAASActive_flg_Inproc/1 -> UnitConverter1161/1
  UnitConverter1161/1 -> VOUTP_CAASActive_flg/1  "VOUTP_CAASActive_flg"
  VVMC_ExtraMSACtrlSta_enum/1 -> VVMC_ExtraMSACtrlSta_enum_Inproc/1  "VVMC_ExtraMSACtrlSta_enum"
  VVMC_ExtraMSACtrlSta_enum_Inproc/1 -> UnitConverter1162/1
  UnitConverter1162/1 -> VOUTP_ExtraMSACtrlSta_enum/1  "VOUTP_ExtraMSACtrlSta_enum"
  VVMC_CalibratedAccX_G/1 -> VVMC_CalibratedAccX_G_Inproc/1  "VVMC_CalibratedAccX_G"
  VVMC_CalibratedAccX_G_Inproc/1 -> UnitConverter1163/1
  UnitConverter1163/1 -> VOUTP_CalibratedAccX_G/1  "VOUTP_CalibratedAccX_G"
  VVMC_CalibratedAccY_G/1 -> VVMC_CalibratedAccY_G_Inproc/1  "VVMC_CalibratedAccY_G"
  VVMC_CalibratedAccY_G_Inproc/1 -> UnitConverter1164/1
  UnitConverter1164/1 -> VOUTP_CalibratedAccY_G/1  "VOUTP_CalibratedAccY_G"
  VVMC_CalibratedAccZ_G/1 -> VVMC_CalibratedAccZ_G_Inproc/1  "VVMC_CalibratedAccZ_G"
  VVMC_CalibratedAccZ_G_Inproc/1 -> UnitConverter1165/1
  UnitConverter1165/1 -> VOUTP_CalibratedAccZ_G/1  "VOUTP_CalibratedAccZ_G"
  VVMC_CalibratedGyroX_Dps/1 -> VVMC_CalibratedGyroX_Dps_Inproc/1  "VVMC_CalibratedGyroX_Dps"
  VVMC_CalibratedGyroX_Dps_Inproc/1 -> UnitConverter1166/1
  UnitConverter1166/1 -> VOUTP_CalibratedGyroX_Dps/1  "VOUTP_CalibratedGyroX_Dps"
  VVMC_CalibratedGyroY_Dps/1 -> VVMC_CalibratedGyroY_Dps_Inproc/1  "VVMC_CalibratedGyroY_Dps"
  VVMC_CalibratedGyroY_Dps_Inproc/1 -> UnitConverter1167/1
  UnitConverter1167/1 -> VOUTP_CalibratedGyroY_Dps/1  "VOUTP_CalibratedGyroY_Dps"
  VVMC_CalibratedGyroZ_Dps/1 -> VVMC_CalibratedGyroZ_Dps_Inproc/1  "VVMC_CalibratedGyroZ_Dps"
  VVMC_CalibratedGyroZ_Dps_Inproc/1 -> UnitConverter1168/1
  UnitConverter1168/1 -> VOUTP_CalibratedGyroZ_Dps/1  "VOUTP_CalibratedGyroZ_Dps"
  VVMC_FDCVMCAPSVRqEPSCtrl_flg/1 -> VVMC_FDCVMCAPSVRqEPSCtrl_flg_Inproc/1  "VVMC_FDCVMCAPSVRqEPSCtrl_flg"
  VVMC_FDCVMCAPSVRqEPSCtrl_flg_Inproc/1 -> UnitConverter1169/1
  UnitConverter1169/1 -> VOUTP_FDCVMCAPSVRqEPSCtrl_flg/1  "VOUTP_FDCVMCAPSVRqEPSCtrl_flg"
  VVMC_FDCVMCAPSAngleTarget_deg/1 -> VVMC_FDCVMCAPSAngleTarget_deg_Inproc/1  "VVMC_FDCVMCAPSAngleTarget_deg"
  VVMC_FDCVMCAPSAngleTarget_deg_Inproc/1 -> UnitConverter1170/1
  UnitConverter1170/1 -> VOUTP_FDCVMCAPSAngleTarget_deg/1  "VOUTP_FDCVMCAPSAngleTarget_deg"
  VVMC_FDCVMCAPSRqEPSCtrl_flg/1 -> VVMC_FDCVMCAPSRqEPSCtrl_flg_Inproc/1  "VVMC_FDCVMCAPSRqEPSCtrl_flg"
  VVMC_FDCVMCAPSRqEPSCtrl_flg_Inproc/1 -> UnitConverter1171/1
  UnitConverter1171/1 -> VOUTP_FDCVMCAPSRqEPSCtrl_flg/1  "VOUTP_FDCVMCAPSRqEPSCtrl_flg"
  VVMC_FDCVMCAngCtrlTqWtGn_pct/1 -> VVMC_FDCVMCAngCtrlTqWtGn_pct_Inproc/1  "VVMC_FDCVMCAngCtrlTqWtGn_pct"
  VVMC_FDCVMCAngCtrlTqWtGn_pct_Inproc/1 -> UnitConverter1172/1
  UnitConverter1172/1 -> VOUTP_FDCVMCAngCtrlTqWtGn_pct/1  "VOUTP_FDCVMCAngCtrlTqWtGn_pct"
  VVMC_FDCVMCDrInpTqBstAct_flg/1 -> VVMC_FDCVMCDrInpTqBstAct_flg_Inproc/1  "VVMC_FDCVMCDrInpTqBstAct_flg"
  VVMC_FDCVMCDrInpTqBstAct_flg_Inproc/1 -> UnitConverter1173/1
  UnitConverter1173/1 -> VOUTP_FDCVMCDrInpTqBstAct_flg/1  "VOUTP_FDCVMCDrInpTqBstAct_flg"
  VVMC_FDCVMCMaxAngCtrlOutTqLim_Nm/1 -> VVMC_FDCVMCMaxAngCtrlOutTqLim_Nm_Inproc/1  "VVMC_FDCVMCMaxAngCtrlOutTqLim_Nm"
  VVMC_FDCVMCMaxAngCtrlOutTqLim_Nm_Inproc/1 -> UnitConverter1174/1
  UnitConverter1174/1 -> VOUTP_FDCVMCMaxAngCtrlOutTqLim_Nm/1  "VOUTP_FDCVMCMaxAngCtrlOutTqLim_Nm"
  VVMC_FDCVMCDrInpTqBstGn_pct/1 -> VVMC_FDCVMCDrInpTqBstGn_pct_Inproc/1  "VVMC_FDCVMCDrInpTqBstGn_pct"
  VVMC_FDCVMCDrInpTqBstGn_pct_Inproc/1 -> UnitConverter1175/1
  UnitConverter1175/1 -> VOUTP_FDCVMCDrInpTqBstGn_pct/1  "VOUTP_FDCVMCDrInpTqBstGn_pct"
  VVMC_VehPitchAngleSta_enum/1 -> VVMC_VehPitchAngleSta_enum_Inproc/1  "VVMC_VehPitchAngleSta_enum"
  VVMC_VehPitchAngleSta_enum_Inproc/1 -> UnitConverter1176/1
  UnitConverter1176/1 -> VOUTP_VehPitchAngleSta_enum/1  "VOUTP_VehPitchAngleSta_enum"
  VVMC_DMSModeCmd_enum/1 -> VVMC_DMSModeCmd_enum_Inproc/1  "VVMC_DMSModeCmd_enum"
  VVMC_DMSModeCmd_enum_Inproc/1 -> UnitConverter1177/1
  UnitConverter1177/1 -> VOUTP_DMSModeCmd_enum/1  "VOUTP_DMSModeCmd_enum"
